simulink model "MPC_Demo_wuguzhang"  (R2024a)
settings: Solver=ode1  StartTime=0.001  StopTime=16  FixedStep=0.001  RelTol=1e-3  EnableMultiTasking=on
model workspace (MAT data in the model file):
  cc = 10
libraries: simulink x3, SignalEditorBlockLib x3, Solver_SF x1, slpidlib x1
(part 2 of 5)

== matlab function MPC_Demo_wuguzhang/区域判断1 ==
  data: sw_angle input; p output; Vx input; beta input; gamma input; miu input
function p = fcn(sw_angle,Vx,beta,gamma,miu)

% C_f=40000;
% C_r=20000;
lr=1.77;
lf=1.18;
Vx_kmh=Vx*3.6;

% Fzf=[0;0;9189.11975037333;9172.89257753388;9169.68008357533;9165.55231050759;9162.51747484095;9160.32031595229;9158.75222397292;9157.63263879663;9156.84242792417;9156.29644556306;9155.92973689187;9155.69322948405;9155.55028107646;9155.47384213415;9155.44421866605;9155.44718649260;9155.47376083021;9155.51788673978;9155.57328214499;9155.63578699923;9155.70821860851;9155.79301339052;9155.88381033351;9155.98423671869;9156.10165075385;9156.23162481467;9156.37616900971;9156.53995716690;9156.71946775849;9156.91602789466;9157.12977373991;9157.35900177799;9157.60378219249;9157.86346416105;9158.13839882949;9158.42758221491;9158.73205404812;9159.05085089054;9159.38485484332;9159.73388891475;9160.09791812571;9160.47713321269;9160.87091175547;9161.27924352332;9161.70131428228;9162.13670893715;9162.25119465208;9162.13371328829;9161.89662615060;9161.62072375802;9161.33377453683;9161.04645701186;9160.75923094872;9160.46913747053;9160.17329178094;9159.86952112061;9159.55619409438;9159.23208125106;9158.89597349374;9158.54671051215;9158.18317131761;9157.80365969706;9157.40862740084;9156.99490198417;9156.56327403121;9156.11090145246;9155.63836107854;9155.14304181031;9154.62545480688;9154.08309726592;9153.51655030897;9152.92339701533;9152.30445793787;9151.65734267787;9150.98324954037;9150.27978025100;9149.54849401502;9148.78705724291;9147.99749395029;9147.17811861429;9146.32961364023;9145.45222801732;9144.54635863102;9143.61254361701;9142.65145880786;9141.66391856333;9140.65087156101;9139.61340091796;9138.55272737068;9137.47019719979;9136.36728195278;9135.24557639213;9134.10679464885;9132.95276535214;9131.78542545848;9130.60681291198;9129.41905838467;9128.22437631368;9127.02505541532;9125.82344880873;9124.62196384518;9123.42305173582;9122.22919703789;9121.04290705517;9119.86670121392;9118.70310047333;9117.55461682614;9116.42374294949;9115.31294206332;9114.22463805584;9113.16120593367;9112.12496265589;9111.11815828058;9110.14296797516;9109.20148309344;9108.29570325586;9107.42753496328;9106.59878144358;9105.81113825995;9105.06619296821;9104.36542108858;9103.71017329634;9103.10168068776;9102.54106265282;9102.02931649768;9101.56731008034;9101.15578484112;9100.79535664774;9100.48651655602;9100.22963286796;9100.02495349837;9099.87260912941;9099.77261648909;9099.72488180259;9099.72920483449;9099.78528310230;9099.89271638063;9100.05100973315;9100.25957652591;9100.51775136266;9100.82479407640;9101.17988031029;9101.58212250571;9102.03058084126;9102.52426045332;9103.06075471025;9103.64370422649;9104.26457543072;9104.93002708322;9105.63124691432;9106.37437100819;9107.15094651253;9107.96665440744;9108.81336807313;9109.69633445555;9110.60777947923;9111.55254145516;9112.52320089777;9113.52418176325;9114.54846792220;9115.60006418080;9116.67234390949;9117.76897492153;9118.88365981330;9120.01975610293;9121.17132428400;9122.33998674980;9123.52500108388;9124.72237568611;9125.93215381899;9127.15390332978;9128.38461103408;9129.62389099137;9130.87122370054;9132.12396531067;9133.38165009435;9134.64240765836;9135.90823350735;9137.17381262979;9138.43979174581;9139.70426262269;9140.96929870188;9142.23006494317;9143.48702667105;9144.73848574261;9145.98490768102;9147.22620961346;9148.45832757067;9149.68193891794;9150.89540854279;9152.09946692694;9153.29250599965;9154.47524214457;9155.64392027933;9156.79931743560;9157.94003328539;9159.06683475530;9160.17836662401;9161.27400846420;9162.35316405762;9163.41667369569;9164.46114963219;9165.48683718486;9166.49460406433;9167.48332197006;9168.45255147890;9169.40187995365;9170.33091814691;9171.23929918847;9172.12667931283;9172.99353321036;9173.83795252978;9174.66047227625;9175.46084439008;9176.23884184991;9176.99425947219;9177.72691520493;9178.43595483914;9179.12262947800;9179.78775597519;9180.42796178708;9181.04481343585;9181.63824556895;9182.20755918311;9182.75411826632;9183.27726127969;9183.77854173865;9184.25494709212;9184.70807679673;9185.13727621803;9185.54416187298;9185.92808386959;9186.29065183294;9186.62907454713;9186.94433319175;9187.23796977694;9187.50952263651;9187.75920730937;9187.98901688782;9188.19487111912;9188.38038274938;9188.54501377853;9188.68905445379;9188.81384810983;9188.91755169024;9189.00155950188;9189.06618384626;9189.11259937906;9189.13946073346;9189.14794628887;9189.13777628342;9189.11241925098;9189.06795546235;9189.00591324040;9188.92803550922;9188.83593797253;9188.72549058666;9188.60040007013;9188.46041109369;9188.30721576260;9188.13868024649;9187.95652438225;9187.76200554478;9187.55387371407;9187.33339566974;9187.10187600015;9186.85798595093;9186.60301610154;9186.33827662843;9186.06246166969;9185.77687505833;9185.48285111761;9185.17902474031;9184.86671645031;9184.54728243101;9184.21926626098;9183.88400875977;9183.54288558470;9183.19434768002;9182.83975307511;9182.48047516083;9182.11489803783;9181.74437300424;9181.37027212888;9180.99094051592;9180.60771723464;9180.22197383280;9179.83198942762;9179.43909316975;9179.04464519644;9178.64685368611;9178.24704018468;9177.84652586583;9177.44353101682;9177.03934194044;9176.63526006740;9176.22946421814;9175.82321710509;9175.41779274990;9175.01133490472;9174.60507199669;9174.20025561793;9173.79497783479;9173.39043897471;9172.98781436236;9172.58523160036;9172.18385145352;9171.78483222679;9171.38629055754;9170.98934733794;9170.59512425417;9170.20173019505;9169.81024293323;9169.42175227098;9169.03433822826;9168.64903632711;9168.26688964956;9167.88600168867;9167.50737979472;9167.13201721731;9166.75801042809;9166.38634069489;9166.01795707694;9165.65098831136;9165.28636482660;9164.92498950869;9164.56500257735;9164.20729114031;9163.85117555379;9163.49995856455;9163.14888329486;9162.79931465538;9162.45246841663;9162.10961063919;9161.76615961809;9161.42524065759;9161.08616205752;9160.75011593112;9160.41447232285;9160.08043677145;9159.74791445801;9159.41784315397;9159.08807917760;9158.75952929936;9158.43209805246;9158.10662407759;9157.78114574669;9157.45647746913;9157.13252640769;9156.80853871300;9156.48758760731;9156.16513450298;9155.84296308772;9155.52033600389;9155.19837927131;9154.87810953021;9154.55589284817;9154.23337689272;9153.90973645886;9153.58628582371;9153.26377321609;9152.93891419752;9152.61317219732;9152.28578068594;9151.95795132814;9151.62889927955;9151.30022042890;9150.96837311411;9150.63438938231;9150.29932776197;9149.96251182374;9149.62384014353;9149.28321573536;9148.94220552383;9148.59676407268;9148.24970801778;9147.90031079378;9147.54849820835;9147.19418663520;9146.83729479511;9146.47774426855;9146.11483883250;9145.75147593996;9145.38349127999;9145.01255952511;9144.63860308171;9144.26156093720;9143.88137876192;9143.49799157288;9143.11077307682;9142.72085029774;9142.32759202698;9141.93096241681;9141.53092481218;9141.12743926432;9140.72211385775;9140.31162106930;9139.89759825382;9139.48002519135;9139.05888807827;9138.63359574431;9138.20530623938;9137.77342355425;9137.33794227599;9136.89885924561;9136.45617769900;9136.00990311330;9135.56004461712;9135.10661820550;9134.64964122897;9134.18913342764;9133.72511700914;9133.25760820384;9132.78663477521;9132.31222436749;9131.83441454675;9131.35324551806;9130.86876037535;9130.38100782374;9129.88949750568;9129.39532089785;9128.89767239263;9128.39670570991;9127.89251075950;9127.38515867153;9126.87471470855;9126.36124182622;9125.84537302540;9125.32417674066;9124.80204764373;9124.27717816046;9123.74965497105;9123.21956094014;9122.68698172171;9122.15058096026;9121.61331428066;9121.07383337722;9120.53223878927;9119.98862662081;9119.44131266172;9118.89448204180;9118.34540452371;9117.79470405791;9117.24248651038;9116.68696570384;9116.13204961098;9115.57650717806;9115.01929674752;9114.46110878973;9113.90003681558;9113.34024166399;9112.78030216564;9112.21931817364;9111.65617063807;9111.09438680595;9110.53288701850;9109.96907858246;9109.40713037513;9108.84544224835;9108.28296668101;9107.72215338406;9107.16196700390;9106.60068042785;9106.04271273031;9105.48506973811;9104.92661874766;9104.37123056312;9103.81779654349;9103.26315877928;9102.71196194787;9102.16289102456;9101.61305434381;9101.06702030360;9100.52343786971;9099.97935565814;9099.43942643879;9098.90226289252;9098.36486096320;9097.83196152604;9097.30211824824;9096.77228000188;9096.24727659962;9095.72561917264;9095.20420159652;9094.68793366034;9094.17529015220;9093.66310946008;9093.15638101205;9092.65354286529;9092.15137876786;9091.65495604354;9091.16267581500;9090.67126815681;9090.18587652965;9089.70486518508;9089.22491013787;9088.75123153871;9088.28215652445;9087.81430271343;9087.35297322559;9086.89645093644;9086.44128776102;9085.99289157789;9085.54949706705;9085.10758108635;9084.67265447228;9084.24290947923;9083.81477096228;9083.39381937667;9082.97821026826;9082.56432062449;9082.15779895098;9081.75676432518;9081.35754565497;9080.96585927416;9080.57978771574;9080.19561128358;9079.81911567907;9079.44834603789;9079.07953403780;9078.71853499425;9078.36335653528;9078.01018133438;9077.66493539057;9077.32381156977;9076.98917087538;9076.65808555041;9076.33475846475;9076.01438207727;9075.70120182675;9075.39221944393;9075.08984879800;9074.79106329829;9074.50016648975;9074.21221493326;9073.93156371471;9073.65510415465;9073.38533279459;9073.11911588335;9072.86086168176;9072.60551250247;9072.35750232993;9072.11362885112;9071.87645854419;9071.64276066227;9071.41703338043;9071.19409503255;9070.97891328353;9070.76668725115;9070.56220363977;9070.36062213141;9070.16676623038;9069.97575309295;9069.79244326532;9069.61191177581;9069.43905674777;9069.26891513290;9069.10642290637;9068.94657150124;9068.79433214199;9068.64465406892;9068.50254538053;9068.36291401772;9068.23080534635;9068.10108627381;9067.97888942288;9067.85902254783;9067.74658937943;9067.63636291736;9067.53349800935;9067.43273609398;9067.33927328873;9067.24781282018;9067.16358810446;9067.08126261596;9067.00610631782;9066.93274315734;9066.86647970992;9066.80190037374;9066.74434910862;9066.68837143878;9066.63934766640;9066.59178496736;9066.55109985993;9066.51176173381;9066.47922312323;9066.44791627699;9066.42332928407;9066.39985700145;9066.38302343676;9066.36718610350;9066.35790536529;9066.34949898786;9066.34756509533;9066.34637995183;9066.35158630174;9066.35742264984;9066.36956516410;9066.38221819143;9066.40109131636;9066.42035472158;9066.44575137466;9066.47141788195;9066.50313069284;9066.53499326668;9066.57281462646;9066.61066580000;9066.65438814625;9066.69802067264;9066.74743681868;9066.79664895074;9066.85157073368;9066.90614847950;9066.96635613957;9067.02610272506;9067.09139120889;9067.15610052285;9067.22626524970;9067.29573416449;9067.37057298801;9067.44460075050;9067.52391389544;9067.60230183596;9067.68589151065;9067.76844305329;9067.85611423211;9067.94263625370;9068.03419653442;9068.12449811267;9068.21975775248;9068.31365072647;9068.41242282498;9068.50972190681;9068.61182246135;9068.71234485189;9068.81759280996;9068.92115997967;9069.02937802419;9069.13581462855;9069.24682393678;9069.35594170585;9069.46956122092;9069.58118996668;9069.69725354845;9069.81123490420;9069.92958647542;9070.04576663818;9070.16625351992;9070.28448141173;9070.40695390077;9070.52708159548;9070.65139339837;9070.77327656374;9070.89928507917;9071.02278247981;9071.15034838708;9071.27532323693;9071.40431155569;9071.53063096107;9071.66091048074;9071.78844521701;9071.91988854349;9072.04851324764;9072.18099685385;9072.31058948489;9072.44399338367;9072.57443651075;9072.70864513503;9072.83982528940;9072.97472688172;9073.10653427471;9073.24202088877;9073.37434956707;9073.51031708560;9073.64306427034;9073.77941195981;9073.91247963514;9074.04911122048;9074.18240497941;9074.31922778111;9074.45265682371;9074.58958182582;9074.72305896922;9074.86000070964;9074.99344173365;9075.13031811045;9075.26364356886;9075.40037659979;9075.53351018252;9075.67002526166;9075.80289412797;9075.93912007685;9076.07165457506;9076.20762618958;9076.33994012781;9076.47560522790;9076.60750110780;9076.74269177696;9076.87405940493;9077.00869981931;9077.13947884137;9077.27351545784;9077.40365414580;9077.53703613674;9077.66648498117;9077.79916388242;9077.92787572113;9078.05980564928;9078.18773600171;9078.31887390679;9078.44598098113;9078.57628584215;9078.70253608326;9078.83198787754;9078.95735993264;9079.08592452977;9079.21037669982;9079.33800991224;9079.46149782897;9079.58815614573;9079.71063706644;9079.83627936397;9079.95771447561;9080.08230305370;9080.20265591840;9080.32615539886;9080.44539183517;9080.56776914034;9080.68585697589;9080.80708096845;9080.92399036489;9081.04403263091;9081.15973660608;9081.27857087922;9081.39304428237;9081.51064642570;9081.62386109856;9081.74019977021;9081.85211637016;9081.96716927885;9082.07778298625;9082.19153551012;9082.30083079064;9082.41326723261;9082.52122888913;9082.63233484261;9082.73894957698;9082.84871271454;9082.95396916875;9083.06237901625;9083.16626764384;9083.27331545418;9083.37582836775;9083.48150700280;9083.58263788106;9083.68694172124;9083.78668576590;9083.88961072053;9083.98796456124;9084.08950789954;9084.18646951440;9084.28662984099;9084.38219852528;9084.48097572667;9084.57515202541;9084.67254720946;9084.76533286020;9084.86134832245;9084.95274627654;9085.04738543560;9085.13739964485;9085.23066696680;9085.31930244827;9085.41120340674;9085.49846616097;9085.58900718734;9085.67490414514;9085.76409258794;9085.84863184481;9085.93646886810;9086.01964538010;9086.10613686697;9086.18797089807;9086.27314322536;9086.35366422064;9086.43754838884;9086.51678787281;9086.59941572272;9086.67740577499;9086.75880971112;9086.83558287214;9086.91579577764;9086.99138515247;9087.07044043382;9087.14500187794;9087.22323484432;9087.29693513225;9087.37417232406;9087.44680699600;9087.52298219243;9087.59455176603;9087.66968800239;9087.74022856174;9087.81436459954;9087.88391378967;9087.95708605231;9088.02567941450;9088.09792271657;9088.16559735393;9088.23694947224;9088.30374016880;9088.37423617995;9088.44017874072;9088.50985445681;9088.57498463890;9088.64387583344;9088.70822931438;9088.77637162225;9088.83998393678;9088.90741285284;9088.97031940026;9089.03707028063;9089.09930631883;9089.16541436883;9089.22701499811;9089.29251525340;9089.35351539604;9089.41844270236;9089.47887708251;9089.54326607469;9089.60316919797;9089.66705428081;9089.72646041517;9089.78987574472;9089.84881890290;9089.91179836935;9089.97031229242;9090.03288950432;9090.09100750218;9090.15321434384;9090.21097115970;9090.27284644192;9090.33026914247;9090.39182317885;9090.44891415001;9090.51014531504;9090.56690107222;9090.62780504086;9090.68422110941;9090.74479309351;9090.80086462530;9090.86109944684;9090.91682119582;9090.97671329867;9091.03207967777;9091.09162320377;9091.14662836125;9091.20581721828;9091.26045509588;9091.31928300664;9091.37354738122;9091.43200792080;9091.48589243780;9091.54397906436;9091.59747726662;9091.65518334896;9091.70828852845;9091.76560556839;9091.81830591656;9091.87521882074;9091.92749726091;9091.98398726991;9092.03582417151;9092.09187091782;9092.14324574108;9092.19882847263;9092.24972067278;9092.30481891756;9092.35520843377;9092.40980235764;9092.45966987547;9092.51374047335;9092.56306756352;9092.61659675861;9092.66536594767;9092.71833664020;9092.76694987876;9092.81989480617;9092.86808876453;9092.92050549057;9092.96810342592;9093.01989279830;9093.06684114055;9093.11798302856;9093.16427323767;9093.21475995923;9093.26038747559;9093.31020490417;9093.35514452025;9093.40429134211;9093.44857733735;9093.49710665222;9093.54080156992;9093.58878030276;9093.63195246381;9093.67944948780;9093.72216778626;9093.76925233330;9093.81158607260;9093.85832780560;9093.90034668310;9093.94681556859;9093.98858948693;9094.03485559718;9094.07645448033;9094.12258783019;9094.16408147988;9094.21015189685;9094.25160987319;9094.29768688632;9094.33917840403;9094.38533114412;9094.42692497715;9094.47322208532;9094.51498647982;9094.56149602333;9094.60349861659;9094.65028801027;9094.69259575552;9094.73973168868;9094.78241078507;9094.82995915415;9094.87307498192;9094.92110082739;9094.96471788756;9095.01328533645;9095.05746719566;9095.10663934031;9095.15144003416;9095.20126893841;9095.24674737198;9095.29729535224;9095.34351519106;9095.39484330569;9095.44186483479;9095.49403270614;9095.54191474796;9095.59498057768;9095.64378135122;9095.69780310035;9095.74757321444;9095.80262426398;9095.85346960418;9095.90961633900;9095.96153288463;9096.01873234039;9096.07165850125;9096.12984089964;9096.18370484932;9096.24279784089;9096.29752785857;9096.35745944501;9096.41298386023;9096.47368188364;9096.52992880802;9096.58880713305;9096.65073967242;9096.70769439850;9096.76772095231;9096.82773074806;9096.88825284891;9096.94905505763;9097.01073497949;9097.07251929632;9097.13478843100;9097.19693679578;9097.25948367104;9097.32184484524;9097.38457525148;9097.44708384530;9097.50993841479;9097.57253255286;9097.63544655280;9097.69805993309;9097.76096667378;9097.82353290400;9097.88636657838;9097.94882050614;9098.01151660772;9098.07379435580;9098.13628961984;9098.19832854112;9098.26056093330;9098.32229962355;9098.38420836398;9098.44558668810;9098.50711227660;9098.56807139169;9098.62915562766;9098.68963800023;9098.75022406668;9098.81018158530;9098.87017361564;9098.92942839833;9098.98869396987;9099.04723669124;9099.10584197675;9099.16377331364;9099.22183299192;9099.27927129301;9099.33690302033;9099.39396438344;9099.45128308826;9099.50808158991;9099.56520077116;9099.62184930654;9099.67888128045;9099.73549144172;9099.79254707600;9099.84922886866;9099.90641732850;9099.96327895499;9100.02070751691;9100.07785521032;9100.13562911006;9100.19316699408;9100.25138929539;9100.30941926024;9100.36818890428;9100.42680316664;9100.48620976831;9100.54550306141;9100.60564528441;9100.66571497179;9100.72668779054;9100.78762729948;9100.84952265743;9100.91142230118;9100.97432906924;9101.03727621998;9101.10128037666;9101.16535951998;9101.23054415542;9101.29583688059;9101.36228218336;9101.42886717296;9101.49665042266;9101.56460344714;9101.63379901040;9101.70319290551;9101.77386569885;9101.84479342531;9101.91709425770;9101.99008630599;9102.06505288356;9102.14052236799;9102.21738698952;9102.29444114421;9102.37277441748;9102.45121861840;9102.53090856501;9102.61066952746;9102.69165076241;9102.77265903962;9102.85485693570;9102.93703467206;9103.02036994155;9103.10363744838;9103.18802998038;9103.27230576112;9103.35736472043;9103.44288307748;9103.52883693248;9103.61520900346;9103.70198116388;9103.78913415925;9103.87665016692;9103.96451277306;9104.05270657283;9104.14121687553;9104.23002946061;9104.31913042516;9104.40850607472;9104.49814285144;9104.58802728667;9104.67814596862;9104.76848552049;9104.85903258592;9104.94977381980;9105.04069588332;9105.13178544139;9105.22302916288;9105.31441372175;9105.40592579971;9105.49755208934;9105.58927929796;9105.68109414329;9105.77298285200;9105.86502467816;9105.95727144182;9106.04973237141;9106.14239697193;9106.23524728144;9106.32826215611;9106.42142033773;9106.51470142641;9106.60808583706;9106.70155457438;9106.79508904889;9106.88867097361;9106.98228232267;9107.07590532060;9107.16952244378;9107.26311642400;9107.35667025140;9107.45016717604;9107.54359070953;9107.63692462611;9107.73015296389;9107.82326002584;9107.91623038111;9108.00904886616;9108.10170058562;9108.19417091310;9108.28644549212;9108.37851023637;9108.47146880858;9108.56466802631;9108.65780385781;9108.75072277300;9108.84333489244;9108.93559715681;9109.02748988741;9109.11900315649;9109.21013163942;9109.30086731147;9109.39163033542;9109.48111772913;9109.57104948012;9109.65968316338;9109.74874378270;9109.83648089723;9109.92464202773;9110.01127918637;9110.09787905307;9110.18261152622;9110.26726474740;9110.35011050194;9110.43298743615;9110.51417714731;9110.59552816735;9110.67530826991;9110.75536777396;9110.83395073786;9110.91291235638;9110.99049688588;9111.06858127637;9111.14539287131;9111.22563877390;9111.29905669339;9111.37886959546;9111.45192459170;9111.53148791288;9111.60439294497;9111.68389985308;9111.75683994196;9111.83647552279;9111.90963184981;9111.98957586428;9112.06312366376;9112.14354945137;9112.21765719014;9112.29873110822;9112.37356020120;9112.45544146430;9112.53114617726;9112.61398678338;9112.69071417765;9112.77465886385;9112.85254876679;9112.93773499093;9113.01691999048;9113.10347793543;9113.18408339511;9113.27213599184;9113.35428008229;9113.44393547413;9113.52792931658;9113.62014516006;9113.70723309837;9113.80265531428;9113.89285087622;9113.99126700142;9114.08426734551;9114.18534199452;9114.28081214436;9114.38421790520;9114.48184229974;9114.58726575906;9114.68673687684;9114.79387016483;9114.89488482556;9115.00342434748;9115.10639421280;9115.21803356981;9115.32373163035;9115.43678897280;9115.54324253492;9115.65675818817;9115.76344261149;9115.87704144072;9115.98367984075;9116.09710569349;9116.20344143075;9116.31643019831;9116.42219932338;9116.53448590031;9116.63942867321;9116.75075489222;9116.85461954785;9116.96473539559;9117.06727820176;9117.17594160895;9117.27692669389;9117.38390346947;9117.48310283418;9117.58816671721;9117.68536029751;9117.78829301737;9117.88327960229;9117.98347412535;9118.07502851036;9118.17143690609;9118.25917099087;9118.35179547629;9118.43589314209;9118.52500449886;9118.60576815830;9118.69165560934;9118.76936245151;9118.85229736205;9118.92721273233;9119.00745869867;9119.07984278309;9119.15765913235;9119.22776786027;9119.30340934826;9119.37149377519;9119.44521000035;9119.51151584834;9119.58355088318;9119.64831224611;9119.71888875423;9119.78229051408;9119.85160870726;9119.91389549335;9119.98219177510;9120.04358960801;9120.11108622362;9120.17181275648;9120.23872423264;9120.29898940402;9120.36552324501;9120.42553015671;9120.49188702999;9120.55183188481;9120.61820546563;9120.67827742679;9120.74485426263;9120.80523535575;9120.87219440930;9120.93306533647;9121.00072909876;9121.06254371323;9121.13119660006;9121.19399939212;9121.26358871951;9121.32728106362;9121.39768930015;9121.46215023415;9121.53325736777;9121.59836867986;9121.67178030971;9121.73984910651;9121.81469362973;9121.88351371954;9121.95874937738;9122.02775600253;9122.10306479959;9122.17210094333;9122.24737890456;9122.31634724850;9122.39148950185;9122.46027857939;9122.53516967457;9122.60366344609;9122.67818739912;9122.74627128960;9122.82031413911;9122.88787563093;9122.96132535402;9123.02825379265;9123.10100020894;9123.16718681728;9123.23912167433;9123.30445967306;9123.37547678109;9123.43986152745;9123.50985691118;9123.57318606083;9123.64205812697;9123.70422980378;9123.77205576467;9123.83357503584;9123.90101001834;9123.96220664999;9124.02926849033;9124.09004522663;9124.15659695408;9124.21680781094;9124.28270432164;9124.34221430027;9124.40732489533;9124.46601013781;9124.53021224465;9124.58795522831;9124.65113194922;9124.70782060935;9124.76986057280;9124.82538841670;9124.88618590817;9124.94045210389;9124.99990711147;9125.05281650636;9125.11083472382;9125.16229783854;9125.21879065283;9125.26872366139;9125.32360812590;9125.37193282203;9125.42513161584;9125.47177536483;9125.52321673922;9125.56811241775;9125.61773013030;9125.66081605520;9125.70854929406;9125.74976914095;9125.79556243961;9125.83486515374;9125.87866829781;9125.91600957773;9125.95724044050;9125.99121170212;9126.02863406286;9126.05880952445;9126.09248847543;9126.11915976076;9126.14947154751;9126.17303182736;9126.20225198389;9126.22570572409;9126.25328347015;9126.27467170389;9126.29996561425;9126.31912378599;9126.34226058284;9126.35947903220;9126.38081487214;9126.39646462860;9126.41635068636;9126.43076450956;9126.44952486201;9126.46301767558;9126.48096294433;9126.49383856383;9126.51126878215;9126.52382043261;9126.54102472172;9126.55353459729;9126.57079085190;9126.58352993698;9126.60110473528;9126.61433276200;9126.63248134612;9126.64644678611;9126.66541306394;9126.68035178511;9126.70036437828;9126.71649071401;9126.73774179251;9126.75574048307;9126.77987819052;9126.80136052105;9126.82900924986;9126.85387895669;9126.88465355073;9126.91240776485;9126.94576558247;9126.97587238470;9127.01129366991;9127.04324860163;9127.08023361112;9127.11354567678;9127.15160508012;9127.18579263687;9127.22444687146;9127.25903858875;9127.29781912561;9127.33235511139;9127.37080533606;9127.40483782437;9127.44251359894;9127.47560743645;9127.51207753775;9127.54676594504;9127.57718616582;9127.61008008743;9127.64290480880;9127.66923857515;9127.69967676543;9127.72773677794;9127.75114364276;9127.77724978939;9127.80023723094;9127.81889873591;9127.83988425756;9127.85752304349;9127.87069694655;9127.88553472756;9127.89582456812;9127.90039207691;9127.90554695929;9127.90618503260;9127.90158294790;9127.89793107813;9127.89037313121;9127.87824970114;9127.86745126833;9127.85337373552;9127.83536292616;9127.81905521835;9127.80002817102;9127.77768057028;9127.75741363961;9127.73496560112;9127.70978324736;9127.68703483868;9127.66262367966;9127.63604318570;9127.61224518740;9127.58881353361;9127.56772391919;9127.54356463785;9127.52263970230;9127.50331849746;9127.48456391293;9127.46178080594;9127.44463156975;9127.42845299543];
% Fzr=[0;0;6232.32629550717;6232.54307244978;6232.91477815521;6233.38563710747;6233.94240655566;6234.56612275444;6235.24014158343;6235.94975524797;6236.68217071639;6237.42636579874;6238.17293314253;6238.91390615096;6239.64258162136;6240.35335056316;6241.04153634985;6241.70324950225;6242.33525801826;6242.93488221073;6243.49989568850;6244.02846586667;6244.51906052474;6244.97039820592;6245.38136911708;6245.75100642514;6246.07846322588;6246.36297904621;6246.60383072906;6246.80036960347;6246.95199291188;6247.05809998131;6247.11813893918;6247.13156377948;6247.09785388636;6247.01652293840;6246.88710479195;6246.70917748785;6246.48234777519;6246.20626625045;6245.88062684790;6245.50516874294;6245.07968149210;6244.60399953319;6244.07800389371;6243.50162311781;6242.87482889067;6242.19763616486;6241.47010421653;6240.69325749782;6239.86887047308;6238.99853701667;6238.08364264689;6237.12533656300;6236.12455959022;6235.08210871880;6233.99868966421;6232.87495516622;6231.71153506660;6230.50905763089;6229.26816569714;6227.98952991147;6226.67385848920;6225.32190441570;6223.93447020719;6222.51241822826;6221.05667963157;6219.56826230537;6218.04825802087;6216.49784870904;6214.91831146876;6213.31102320262;6211.67746371988;6210.01921840042;6208.33797977737;6206.63554855827;6204.91383349772;6203.17485035373;6201.42072042279;6199.65366783259;6197.87601594993;6196.09018298240;6194.29867649363;6192.50408715584;6190.70908153284;6188.91639406113;6187.12881866016;6185.34920076739;6183.58043063022;6181.82543772309;6180.08718398131;6178.36865294418;6176.67283452149;6175.00270757929;6173.36122316766;6171.75129009974;6170.17576309679;6168.63743273341;6167.13901626998;6165.68314878347;6164.27237436612;6162.90913737779;6161.59577384296;6160.33450311111;6159.12741990012;6157.97648683183;6156.88352755229;6155.85022051378;6154.87809348015;6153.96851880348;6153.12270950579;6152.34171619001;6151.62642479179;6150.97755598273;6150.39566203877;6149.88112879779;6149.43417657454;6149.05486469573;6148.74309027663;6148.49862455822;6148.32109516155;6148.20994913313;6148.16450785900;6148.18398907915;6148.26733216398;6148.41341271497;6148.62099076394;6148.88871686543;6149.21513895527;6149.59870939931;6150.03779222830;6150.53067144950;6151.07555547907;6151.67058539835;6152.31384611903;6153.00337003910;6153.73714659725;6154.51312451647;6155.32922586525;6156.18334687456;6157.07336607688;6157.99715026078;6158.95256019230;6159.93759583914;6160.95016315556;6161.98819906054;6163.04965966232;6164.13250628364;6165.23479089180;6166.35433364972;6167.48900944461;6168.63677935195;6169.79565436234;6170.96368243236;6172.13896926358;6173.31967359229;6174.50400719840;6175.69023494123;6176.87667516223;6178.06170505400;6179.24374582456;6180.42127639731;6181.59284071226;6182.75703800449;6183.91252366763;6185.05801005314;6186.19232015262;6187.31449596826;6188.42344096218;6189.51819705809;6190.59783935364;6191.66147534015;6192.70824818866;6193.73746774156;6194.74808164146;6195.73917056629;6196.70993629329;6197.65964820737;6198.58764042383;6199.49330867453;6200.37610767006;6201.23554866657;6202.07119730098;6202.88267141960;6203.66963908356;6204.43181665521;6205.16896713034;6205.88089828291;6206.56746105420;6207.22854790898;6207.86409122286;6208.47406187048;6209.05852403975;6209.61775614362;6210.15184926026;6210.66102424303;6211.14551327852;6211.60555333665;6212.04139013678;6212.45328440392;6212.84155312069;6213.20654460609;6213.54818451946;6213.86668640068;6214.16229575237;6214.43529544672;6214.68600186793;6214.91476162182;6215.12194859209;6215.30796126885;6215.47322036576;6215.61816664606;6215.74325886941;6215.84897195107;6215.93579520111;6216.00423089911;6216.05479273188;6216.08800523180;6216.10439905011;6216.10451413064;6216.08889765087;6216.05810244017;6216.01275759639;6215.95361368156;6215.88121559152;6215.79621429256;6215.69924316657;6215.59091770681;6215.47183771977;6215.34258908201;6215.20374627649;6215.05586918862;6214.89965852940;6214.73545381670;6214.56360571013;6214.38456114853;6214.19877595683;6214.00671218816;6213.80883540318;6213.60561253909;6213.39751008011;6213.18499242210;6212.96852054834;6212.74855080405;6212.52553404491;6212.29991470726;6212.07213000898;6211.84260932788;6211.61177358329;6211.38003468928;6211.14779503167;6210.91544696403;6210.68337256638;6210.45194316022;6210.22151902998;6209.99246020095;6209.76532049044;6209.54036367215;6209.31796855286;6209.09849329397;6208.88227042621;6208.66960906184;6208.46079678628;6208.25610126088;6208.05577161734;6207.86003958897;6207.66912039667;6207.48334009407;6207.30278886318;6207.12744366031;6206.95740495393;6206.79277311370;6206.63364715094;6206.48012346085;6206.33229481613;6206.19024963394;6206.05407159773;6205.92383925885;6205.79962581958;6205.68149914694;6205.56952166886;6205.46375038059;6205.36423695986;6205.27102775488;6205.18416394500;6205.10368174323;6205.02961240169;6204.96198242721;6204.90081388743;6204.84612444751;6204.79792752491;6204.75640587035;6204.72153470589;6204.69334033636;6204.67186727776;6204.65714568721;6204.64919341197;6204.64801780378;6204.65361693010;6204.66598083127;6204.68509275114;6204.71092991295;6204.74346222326;6204.78265904750;6204.82853175901;6204.88115179724;6204.94020928045;6205.00561803686;6205.07729616520;6205.15516841437;6205.23916465508;6205.32921878341;6205.42526809591;6205.52725250011;6205.63511397390;6205.74879629675;6205.86824459694;6205.99340496484;6206.12422447159;6206.26065087089;6206.40263250683;6206.55011830475;6206.70305765397;6206.86139991053;6207.02509507597;6207.19409348994;6207.36834579852;6207.54780278749;6207.73253047355;6207.92249492935;6208.11763883793;6208.31795073179;6208.52341070259;6208.73399190606;6208.94966184019;6209.17038339978;6209.39611572623;6209.62681502371;6209.86243513669;6210.10292801924;6210.34824426433;6210.59833324054;6210.85314375951;6211.11262415044;6211.37680024137;6211.64563275382;6211.91889712103;6212.19651273494;6212.47840530174;6212.76450670357;6213.05475415533;6213.34908918386;6213.64745348996;6213.94980192073;6214.25608177929;6214.56624613090;6214.88024984879;6215.19804927543;6215.51960207411;6215.84486702092;6216.17380395790;6216.50637360705;6216.84253743073;6217.18225755812;6217.52549661361;6217.87221777134;6218.22238457463;6218.57596079207;6218.93291029659;6219.29333120175;6219.65712566143;6220.02428343472;6220.39479307441;6220.76863697282;6221.14579243785;6221.52623254301;6221.90992684291;6222.29684187085;6222.68694153615;6223.08018756314;6223.47653983935;6223.87595670669;6224.27839346810;6224.68380823475;6225.09215639671;6225.50339129141;6225.91746635481;6226.33433376693;6226.75394475990;6227.17639939794;6227.60145517817;6228.02903561687;6228.45907232249;6228.89150075567;6229.32625944927;6229.76328931003;6230.20253303801;6230.64393463598;6231.08743904390;6231.53299179711;6231.98053890938;6232.43002665144;6232.88140140623;6233.33460955766;6233.78959736315;6234.24631086481;6234.70469575265;6235.16469738838;6235.62626071425;6236.08933015638;6236.55384966182;6237.01976267974;6237.48701215796;6237.95554053729;6238.42528970225;6238.89628911481;6239.36844916086;6239.84171937130;6240.31605699245;6240.79141452918;6241.26774000497;6241.74497774611;6242.22306900801;6242.70195006769;6243.18155353923;6243.66180950138;6244.14264587439;6244.62398889832;6245.10576349998;6245.58789362644;6246.07030256871;6246.55291324194;6247.03564826367;6247.51843002977;6248.00118084498;6248.48382300004;6248.96627882496;6249.44847078858;6249.93032142681;6250.41175333223;6250.89272200385;6251.37318787692;6251.85296928028;6252.33197760981;6252.81012691231;6253.28733434283;6253.76351960102;6254.23860456611;6254.71251292996;6255.18516994540;6255.65650230787;6256.12643798495;6256.59490618762;6257.06183723674;6257.52716244149;6257.99081412096;6258.45272452139;6258.91282390173;6259.37104244001;6259.82731019489;6260.28155752044;6260.73371515528;6261.18371458789;6261.63148827798;6262.07696955473;6262.52009287576;6262.96079393272;6263.39900953590;6263.83471509219;6264.26786614187;6264.69838981181;6265.12624084926;6265.55137213252;6265.97373512237;6266.39328053268;6266.80995873773;6267.22371991912;6267.63451452720;6268.04229350587;6268.44700828650;6268.84861118627;6269.24705538980;6269.64229499736;6270.03428526246;6270.42298257896;6270.80834446780;6271.19032977736;6271.56889863779;6271.94401241881;6272.31563391109;6272.68372725921;6273.04825790343;6273.40919274914;6273.76650008666;6274.12014952336;6274.47011214560;6274.81636043000;6275.15886816665;6275.49761061829;6275.83256442392;6276.16370752940;6276.49101932996;6276.81448060413;6277.13407345579;6277.44984826445;6277.76171274427;6278.06963857261;6278.37360695119;6278.67360203923;6278.96961111902;6279.26162348542;6279.54963035640;6279.83362470823;6280.11360125645;6280.38955625502;6280.66148735875;6280.92939369905;6281.19327571323;6281.45313503489;6281.70897459717;6281.96079847795;6282.20861180562;6282.45242087643;6282.69223300835;6282.92805645465;6283.15990052961;6283.38777546617;6283.61169233613;6283.83166319343;6284.04770080793;6284.25981889731;6284.46803187985;6284.67235502283;6284.87280422751;6285.06941331865;6285.26221716409;6285.45122125625;6285.63645173386;6285.81793359921;6285.99569077622;6286.16974663266;6286.34012390789;6286.50684520593;6286.66993287453;6286.82940930867;6286.98529683282;6287.13761802172;6287.28639544274;6287.43165198542;6287.57341065358;6287.71169477161;6287.84652780797;6287.97793358862;6288.10593608951;6288.23055965142;6288.35182876148;6288.46976826484;6288.58440314260;6288.69575871935;6288.80386042444;6288.90873400216;6289.01040528240;6289.10890039295;6289.20424553008;6289.29646717135;6289.38559184397;6289.47164633870;6289.55465747187;6289.63465220569;6289.71165746974;6289.78570043891;6289.85680830099;6289.92500847689;6289.99032838028;6290.05279563342;6290.11243782368;6290.16928272419;6290.22335805077;6290.27469168612;6290.32331143623;6290.36924525640;6290.41252100906;6290.45316669306;6290.49121019948;6290.52667954363;6290.55960261971;6290.59000758036;6290.61792222515;6290.64337423408;6290.66639118118;6290.68700070156;6290.70523027147;6290.72110746011;6290.73466290452;6290.74595376259;6290.75496624998;6290.76172479797;6290.76625415103;6290.76857984531;6290.76872782054;6290.76672455514;6290.76259671958;6290.75637135298;6290.74807554510;6290.73773664073;6290.72538194170;6290.71103892849;6290.69473497384;6290.67649757655;6290.65635408265;6290.63433192725;6290.61045836024;6290.58476069396;6290.55726608694;6290.52800164533;6290.49699435946;6290.46427110637;6290.42985865268;6290.39378364350;6290.35607260431;6290.31675193173;6290.27584789545;6290.23338662897;6290.18939413225;6290.14389626197;6290.09691873331;6290.04848711201;6289.99862681723;6289.94736311254;6289.89472111094;6289.84072576600;6289.78540187655;6289.72877407842;6289.67086684948;6289.61170450082;6289.55131118206;6289.48971087131;6289.42692738282;6289.36298435750;6289.29790526964;6289.23171341796;6289.16443193315;6289.09608946626;6289.02671521977;6288.95632698547;6288.88494971010;6288.81260756095;6288.73932400563;6288.66512190818;6288.59002361436;6288.51405101500;6288.43722560424;6288.35956852014;6288.28110058455;6288.20184232814;6288.12181401907;6288.04103567767;6287.95952709623;6287.87730784891;6287.79439730641;6287.71081464059;6287.62657883582;6287.54170869023;6287.45622282519;6287.37013968454;6287.28347754162;6287.19625449585;6287.10848847900;6287.02019725335;6286.93139841737;6286.84210940240;6286.75234747824;6286.66212974914;6286.57147315903;6286.48039448727;6286.38891035384;6286.29703721294;6286.20479135888;6286.11218892106;6286.01924586829;6285.92597800448;6285.83240097389;6285.73853025586;6285.64438117035;6285.54996887229;6285.45530835669;6285.36041445175;6285.26530182567;6285.16998498050;6285.07447825804;6284.97879583332;6284.88295172015;6284.78695976560;6284.69083365563;6284.59458690948;6284.49823287987;6284.40178458428;6284.30525475956;6284.20865601812;6284.11200085529;6284.01530164610;6283.91857064800;6283.82181998362;6283.72506163852;6283.62830744792;6283.53156909845;6283.43485811912;6283.33818588476;6283.24156360785;6283.14500234352;6283.04851298186;6282.95210625356;6282.85579272274;6282.75958279165;6282.66348669293;6282.56751448412;6282.47167603779;6282.37598105310;6282.28043905458;6282.18505940504;6282.08985130338;6281.99482379558;6281.89998576887;6281.80534596204;6281.71091296000;6281.61669520197;6281.52270097453;6281.42893842088;6281.33541553385;6281.24214016406;6281.14912001262;6281.05636263775;6280.96387544931;6280.87166571557;6280.77974055655;6280.68810695194;6280.59677173309;6280.50574159073;6280.41502306644;6280.32462252283;6280.23454614690;6280.14479997278;6280.05538987084;6279.96632155992;6279.87760060292;6279.78923241860;6279.70122227596;6279.61357530482;6279.52629648856;6279.43939067409;6279.35286256555;6279.26671673308;6279.18095760586;6279.09558948113;6279.01061651689;6278.92604274095;6278.84187204314;6278.75810818491;6278.67475479055;6278.59181535654;6278.50929324396;6278.42719168821;6278.34551379083;6278.26426252938;6278.18344074960;6278.10305117463;6278.02309639763;6277.94357889133;6277.86450099967;6277.78586494736;6277.70767283147;6277.62992663216;6277.55262820455;6277.47577928850;6277.39938150098;6277.32343634598;6277.24794520649;6277.17290935492;6277.09832994447;6277.02420801956;6276.95054450656;6276.87734022285;6276.80459587694;6276.73231206936;6276.66048927789;6276.58912785949;6276.51822803484;6276.44778989298;6276.37781337833;6276.30829829829;6276.23924431109;6276.17065093583;6276.10251754240;6276.03484336233;6275.96762747938;6275.90086884084;6275.83456624897;6275.76871819920;6275.70332269923;6275.63837774298;6275.57388123595;6275.50983103520;6275.44622494243;6275.38306069719;6275.32033595544;6275.25804829134;6275.19619518114;6275.13477400952;6275.07378205688;6275.01321650643;6274.95307440552;6274.89335268587;6274.83404816198;6274.77515754311;6274.71667742726;6274.65860431509;6274.60093460263;6274.54366459507;6274.48679049893;6274.43030843573;6274.37421443391;6274.31850444249;6274.26317432256;6274.20821986106;6274.15363676203;6274.09942066030;6274.04556711275;6273.99207161192;6273.93892957688;6273.88613636724;6273.83368727372;6273.78157753202;6273.72980231344;6273.67835673868;6273.62723586854;6273.57643471739;6273.52594824390;6273.47577136461;6273.42589894426;6273.37632580988;6273.32704674028;6273.27805648116;6273.22934974096;6273.18092120742;6273.13276555093;6273.08487745157;6273.03725160201;6272.98988273380;6272.94276561580;6272.89589507562;6272.84926599378;6272.80287332236;6272.75671207613;6272.71077734880;6272.66506430281;6272.61956818385;6272.57428430938;6272.52920808268;6272.48433497985;6272.43966056376;6272.39518047041;6272.35089042227;6272.30678621437;6272.26286372733;6272.21911891313;6272.17554780820;6272.13214651861;6272.08891123305;6272.04583820836;6272.00292377693;6271.96016432695;6271.91755631405;6271.87509624666;6271.83278069923;6271.79060629860;6271.74856973777;6271.70666776237;6271.66489718446;6271.62325486870;6271.58173774555;6271.54034279711;6271.49906707032;6271.45790766225;6271.41686173290;6271.37592649028;6271.33509920335;6271.29437718666;6271.25376129659;6271.21325674296;6271.17285496884;6271.13255502899;6271.09235560243;6271.05225509759;6271.01225175727;6270.97234367883;6270.93252886056;6270.89280521203;6270.85317058796;6270.81362279045;6270.77415958630;6270.73477870423;6270.69547783496;6270.65625459909;6270.61710654071;6270.57803109363;6270.53902558097;6270.50008718961;6270.46121297648;6270.42239984851;6270.38364457410;6270.34494376645;6270.30629389807;6270.26769128659;6270.22913211127;6270.19061240011;6270.15212804831;6270.11367480581;6270.07524829671;6270.03684400788;6269.99845730846;6269.96008343935;6269.92171753269;6269.88335460157;6269.84498956030;6269.80661721370;6269.76823227761;6269.72982936841;6269.69140302334;6269.65294769033;6269.61445774811;6269.57592749597;6269.53735117401;6269.49872295257;6269.46003695284;6269.42128723557;6269.38246782215;6269.34357268304;6269.30459575839;6269.26553094686;6269.22639616321;6269.18716676098;6269.14782437929;6269.10836075743;6269.06876810558;6269.02903902178;6268.98916643421;6268.94914352666;6268.90896370843;6268.86862056025;6268.82810814584;6268.78742004619;6268.74654988618;6268.70549143248;6268.66423852249;6268.62278504707;6268.58112499840;6268.53925249409;6268.49716183830;6268.45484754418;6268.41230438232;6268.36952738691;6268.32651188998;6268.28325351548;6268.23974820507;6268.19599220470;6268.15198208483;6268.10771472277;6268.06318731914;6268.01839737926;6267.97334272089;6267.92802142481;6267.88243195987;6267.83657302047;6267.79044359248;6267.74404254163;6267.69736825140;6267.65041960255;6267.60319589310;6267.55569683391;6267.50792259171;6267.45987369186;6267.41155102878;6267.36295578563;6267.31408945722;6267.26495377970;6267.21555076160;6267.16588261908;6267.11595181103;6267.06576097763;6267.01531297771;6266.96461082963;6266.91365775063;6266.86245709870;6266.81101241325;6266.75932735831;6266.70740576405;6266.65525157035;6266.60286886927;6266.55026184942;6266.49743483852;6266.44439224844;6266.39113861798;6266.33767855883;6266.28401679810;6266.23015811482;6266.17610745062;6266.12186985349;6266.06745046485;6266.01285440660;6265.95808676506;6265.90315248829;6265.84805639209;6265.79280307937;6265.73739696317;6265.68184220050;6265.62614272608;6265.57030219549;6265.51432402612;6265.45821134590;6265.40196703873;6265.34559369759;6265.28909367301;6265.23246902838;6265.17572159093;6265.11885290852;6265.06186430194;6265.00475682277;6264.94753130700;6264.89018833293;6264.83272827562;6264.77517541802;6264.71752346223;6264.65977091773;6264.60192195165;6264.54397934321;6264.48594476488;6264.42781892011;6264.36960174224;6264.31129247283;6264.25288981136;6264.19439195338;6264.13579670755;6264.07710150720;6264.01830350624;6263.95939957309;6263.90038637201;6263.84126034594;6263.78201778792;6263.72265481620;6263.66316743977;6263.60355152764;6263.54380287035;6263.48391714580;6263.42388998595;6263.36371690219;6263.30339333629;6263.24291415181;6263.18230157418;6263.12155010616;6263.06061447383;6262.99948566888;6262.93815597893;6262.87661884862;6262.81486875200;6262.75290100432;6262.69071169388;6262.62829754305;6262.56565587848;6262.50278452259;6262.43968179594;6262.37634754298;6262.31278108416;6262.24898193827;6262.18495002186;6262.12068538995;6262.05618829470;6261.99145917929;6261.92649868517;6261.86130765314;6261.79588713032;6261.73023837047;6261.66436283090;6261.59826216851;6261.53193823391;6261.46539306524;6261.39862888154;6261.33164807564;6261.26445320717;6261.19704699564;6261.12943231355;6261.06161217944;6260.99358975144;6260.92536832053;6260.85695130410;6260.78834223979;6260.71954477934;6260.65056268231;6260.58139981049;6260.51206012192;6260.44254766556;6260.37286656640;6260.30302085490;6260.23301437752;6260.16285080973;6260.09253367361;6260.02206636792;6259.95145219567;6259.88069438498;6259.80979610436;6259.73876047454;6259.66759057694;6259.59628946008;6259.52486014451;6259.45330562613;6259.38162887912;6259.30983285746;6259.23792049664;6259.16589471422;6259.09375841049;6259.02151446863;6258.94916575504;6258.87671511918;6258.80416539325;6258.73151939255;6258.65877991475;6258.58594974021;6258.51303163151;6258.44002833355;6258.36694252093;6258.29377508372;6258.22052681016;6258.14719855508;6258.07379151729;6258.00033579600;6257.92683533752;6257.85328475756;6257.77969337212;6257.70606887251;6257.63241764065;6257.55874499085;6257.48505536380;6257.41135250652;6257.33763957118;6257.26391926075;6257.19019387382;6257.11646542047;6257.04273593874;6256.96900804130;6256.89528472683;6256.82156936869;6256.74786554081;6256.67417693346;6256.60050721413;6256.52685999703;6256.45327968724;6256.37976653188;6256.30627063168;6256.23278964525;6256.15932212628;6256.08586745744;6256.01242560079;6255.93899697208;6255.86558227439;6255.79218246333;6255.71879854776;6255.64543161505;6255.57208272250;6255.49875291733;6255.42544314964;6255.35215430944;6255.27888715228;6255.20564234633;6255.13242040684;6255.05922174997;6254.98604663282;6254.91289521194;6254.83976748696;6254.76666336148;6254.69358258941;6254.62052483730;6254.54748963205;6254.47447642415;6254.40148453631;6254.32851322686;6254.25556163896;6254.18262886428;6254.10971389175;6254.03681567136;6253.96393306347;6253.89106490278;6253.81820959224;6253.74536442604;6253.67252584675;6253.59969049341;6253.52685373359;6253.45400874680;6253.38114950577;6253.30826992533;6253.23536412252;6253.16242660245;6253.08945229295;6253.01643666231;6252.94337570550;6252.87026602530;6252.79710479200;6252.72388980375;6252.65061796532;6252.57728352499;6252.50388160929;6252.43040779806;6252.35685844727;6252.28323082791;6252.20952300147;6252.13573382559;6252.06186285553;6251.98791036248;6251.91387724685;6251.83976506696;6251.76557595879;6251.69131266717;6251.61697846823;6251.54257720246;6251.46811319894;6251.39359130913;6251.31901683308;6251.24439555394;6251.16973366545;6251.09503780731;6251.02031499340;6250.94557264812;6250.87081853522;6250.79606079464;6250.72130788476;6250.64656929842;6250.57186459856;6250.49724453050;6250.42269577640;6250.34823925527;6250.27389461505;6250.19967977830;6250.12561109225;6250.05170354864;6249.97797087554;6249.90442570806;6249.83107963803;6249.75794334902;6249.68502663851;6249.61233852926;6249.53988727288;6249.46768044597;6249.39572494172;6249.32402705536;6249.25259246823;6249.18148578411;6249.11067683111;6249.04012718220;6248.96983487982;6248.89979883299;6248.83001861353;6248.76049430138;6248.69122627961;6248.62221515488;6248.55346161217;6248.48496638189;6248.41673013279;6248.34875346980;6248.28103685211;6248.21358061114;6248.14638488445;6248.07944964701;6248.01277465638;6247.94635949156;6247.88020350545;6247.81430587031;6247.74866552833;6247.68328100491;6247.61815048528;6247.55327193381;6247.48864316703;6247.42426200793;6247.36012633006;6247.29623416966;6247.23258373471;6247.16917348780;6247.10600205896;6247.04306546816;6246.98036005101;6246.91788253400;6246.85563050429;6246.79360252262;6246.73179797108;6246.67021698829;6246.60886033268;6246.54772934508;6246.48682584302;6246.42615211103;6246.36571081532;6246.30550500861;6246.24553805539;6246.18581364525;6246.12633572526;6246.06710851825;6246.00813646063;6245.94942422434;6245.89097665797;6245.83279881145;6245.77489587953;6245.71727322815;6245.65993633712;6245.60289082666;6245.54614240136;6245.48969687611;6245.43356012172;6245.37773809208;6245.32223676423;6245.26706185460;6245.21221915753;6245.15771516265;6245.10355301750;6245.04973643576;6244.99626835034;6244.94315120492;6244.89038701381;6244.83797747982;6244.78592401749;6244.73422784170;6244.68288996896;6244.63191128799;6244.58129254682;6244.53103441172;6244.48113744517;6244.43160215684;6244.38242897545;6244.33361829459;6244.28517044092;6244.23708571609;6244.18936436242;6244.14200660305;6244.09501260557;6244.04838252071;6244.00211644547;6243.95621446033;6243.91067659209;6243.86550285051;6243.82069319094;6243.77624755042;6243.73216581058;6243.68844783304;6243.64509342286;6243.60210236378;6243.55947438133;6243.51720917850;6243.47530639916;6243.43376566306;6243.39258655858;6243.35176961919;6243.31131656345;6243.27123014270;6243.23151384722;6243.19217163671;6243.15320764119;6243.11462599106;6243.07643054709;6243.03862154957;6243.00119886826;6242.96416214070;6242.92751100077;6242.89124552098;6242.85536558838;6242.81987124963;6242.78476211298;6242.75003771520;6242.71569700706;6242.68173875165;6242.64816105061;6242.61496176395;6242.58213806047;6242.54968684810;6242.51760434061;6242.48588649298;6242.45452858104;6242.42352563752;6242.39287204137;6242.36256195332;6242.33258891219;6242.30294626811;6242.27362678487;6242.24462307024;6242.21592718251;6242.18754405276;6242.15946604679;6242.13168072572;6242.10418199784;6242.07696285127;6242.05005513092;6242.02341148260;6241.99700302656;6241.97081260203;6241.94482283814;6241.91901687717;6241.89337821371;6241.86789125383;6241.84254106062;6241.81731383184;6241.79219658705;6241.76717759462;6241.74224602500;6241.71739234393;6241.69260794518;6241.66788551944;6241.64321867566;6241.61860229232;6241.59403213254;6241.56950518274;6241.54501926564;6241.52057336867;6241.49616725816;6241.47180179942;6241.44747857267;6241.42320018361;6241.39896997049;6241.37479203109;6241.35067127434;6241.32661330584;6241.30262436348;6241.27871141725;6241.25488200706;6241.23114422485;6241.20750679467;6241.18397889029;6241.16057015758;6241.13729075553;6241.11415164200;6241.09116607899;6241.06834897359;6241.04571638914;6241.02328499495;6241.00107157523;6240.97909246018;6240.95736323232;6240.93589849854;6240.91471171325;6240.89381485797;6240.87321858606;6240.85293202066;6240.83296258522;6240.81331621681;6240.79399723080;6240.77500819053;6240.75635020160;6240.73802279270;6240.72002379126;6240.70234965851;6240.68499534902;6240.66795169927;6240.65120637074;6240.63474630328;6240.61855777230;6240.60262663825;6240.58693831134;6240.57147769154;6240.55622904970];
% 
% alpha_fy=(-0.3+0.6/1462:0.6/1462:0.3);
alpha_ry=(-0.25+0.5/1462:0.5/1462:0.25);

% %定义矩阵分配内存
% Fyfy=zeros(1,length(alpha_fy));
% Fyry=zeros(1,length(alpha_ry));
% C1=zeros(1,length(alpha_fy)-1);C3=zeros(1,length(alpha_ry)-1);
% Cfl=zeros(1,258);Crl=zeros(1,258);
% 
% 
% for iif=1:length(alpha_fy)
%     if abs(alpha_fy(iif))<atan((3*miu*Fzf(iif))/C_f)
%     Fyfy(iif)=(-C_f*alpha_fy(iif)+(C_f)^2/(3*miu*Fzf(iif))*abs(alpha_fy(iif))*alpha_fy(iif)-(C_f)^3/(27*miu^2*Fzf(iif)^2)*(alpha_fy(iif))^3);
%     else
%         Fyfy(iif)=-miu*Fzf(iif)*sign(alpha_fy(iif));
%     end
% end
% for iir=1:length(alpha_ry)
%     if abs(alpha_ry(iir))<atan((3*miu*Fzr(iir))/C_r)
%     Fyry(iir)=(-C_r*alpha_ry(iir)+(C_r)^2/(3*miu*Fzr(iir))*abs(alpha_ry(iir))*alpha_ry(iir)-(C_r)^3/(27*miu^2*Fzr(iir)^2)*(alpha_ry(iir))^3);
%     else
%          Fyry(iir)=-miu*Fzr(iir)*sign(alpha_ry(iir));
%     end
% end
% 
% for x1=1:length(alpha_fy)-1
% C1(x1)=(Fyfy(x1+1)-Fyfy(x1))/(-(alpha_fy(x1+1))-(-alpha_fy(x1)));
% Cfll=C1';
% end
% for x3=1:length(alpha_ry)-1
% C3(x3)=(Fyry(x3+1)-Fyry(x3))/(-(alpha_ry(x3+1))-(-alpha_ry(x3)));
% Crll=C3';
% end
% for aaf=1:258
%   Cfl(aaf)=Cfll(5*aaf);
% end
% for aar=1:258
%    Crl(aar)=Crll(5*aar); 
% end

alpharl=[alpha_ry];


% for i=1:a 
%         for k=1:c 
%                 if Cfl(i)>(-(lr*(Crl(k))*1430*(Vx^2)))/(2*(Crl(k))*((lf+lr)^2)-1430*(Vx^2)*lf)
%                     aa=[Cfl(i) Crl(k)];
%                     cc=[-alphafl(5*i+1) -alpharl(5*k+1)];
%                     A=[A;aa];
%                     C=[C;cc];
%                 else
%                     bb=[Cfl(i) Crl(k)];
%                     dd=[-alphafl(5*i+1) -alpharl(5*k+1)];
%                     B=[B;bb];
%                     D=[D;dd];
%                 end
%         end
% end

% Cf=B(:,1);
% Cr=B(:,2);
% osCf=[];
% osCr=[];
% oalphaf=[];
% oalphar=[];
% usCf=[];
% usCr=[];
% ualphaf=[];
% ualphar=[];
beta1_right=zeros(1,length(alpharl));
gamma1_right=zeros(1,length(alpharl));

% for p=1:length(Cf)
%     if lf*Cf(p)-lr*Cr(p)>0
%         osCf=[osCf;Cf(p)];%%婊¤冻杩囧害杞悜鏉′欢鐨凜f
%         osCr=[osCr;Cr(p)];%%婊¤冻杩囧害杞悜鏉′欢鐨凜r
%         oalphaf=[oalphaf;Alphaf(p)];%%婊¤冻杩囧害杞悜鏉′欢鐨刟lphaf
%         oalphar=[oalphar;Alphar(p)];%%婊¤冻杩囧害杞悜鏉′欢鐨刟lphar
%     else
%         usCf=[usCf;Cf(p)];%%婊¤冻涓嶈冻杞悜鏉′欢鐨凜f
%         usCr=[usCr;Cr(p)];%%婊¤冻涓嶈冻杞悜鏉′欢鐨凜r
%         ualphaf=[ualphaf;Alphaf(p)];%%婊¤冻涓嶈冻杞悜鏉′欢鐨刟lphaf
%         ualphar=[ualphar;Alphar(p)];%%婊¤冻涓嶈冻杞悜鏉′欢鐨刟lphar
%     end
% end    
kekoalphaf=-0.3;%%%%%鍜岄�鎷╃殑鍓嶈疆渚у亸瑙掔殑澶у皬鏈夊叧

%%
if Vx_kmh <= 52.5
%% 外区域
for n=1:length(alpharl)
    if abs(alpharl(n))<abs(kekoalphaf)%%鐢ㄤ笉瓒宠浆鍚戞椂鍓嶅悗杞晶鍋忚鐨勫ぇ灏忓叧绯荤瓫閫夊悎閫傜殑
    beta1_right(n)=((sw_angle-kekoalphaf)*lr-lf*alpharl(n))/(lf+lr);
    gamma1_right(n)=((sw_angle-kekoalphaf+alpharl(n))*Vx)/(lf+lr);
    end
end

   beta11_50_right_down=beta1_right(1);
   gamma11_50_right_down=gamma1_right(1);
   beta1n_50_right_up=beta1_right(length(beta1_right));
   gamma1n_50_right_up=gamma1_right(length(gamma1_right));
   
    centerx_50=beta1n_50_right_up-0.0829;
    centery_50=gamma1n_50_right_up-2.8718;
   
    beta1d1_50_left_up=2*centerx_50-beta1_right(1);
    gamma1d1_50_left_up=2*centery_50-gamma1_right(1);
    beta1dn_50_left_down=2*centerx_50-beta1_right(length(beta1_right));
    gamma1dn_50_left_down=2*centery_50-gamma1_right(length(gamma1_right));
    
g1=2.1343+gamma1dn_50_left_down;%璁＄畻ogamma2_down(1)-gamma1dn_50_left_down=锛熶綔涓哄墠闈㈢殑涓?釜鍔犳暟;
b1=0.0504+beta1dn_50_left_down;%obeta2_down(1)-beta1dn_50_left_down=锛?
g2=0.8857+g1;%ogamma2_down(length(ogamma2_down))-ogamma2_down(1)=锛?
b2=0.0993+b1;%obeta2_down(length(obeta2_down))-obeta2_down(1)=锛?
g3=2*centery_50-g1;%%-g1
b3=2*centerx_50-b1;%%-b1
g4=2*centery_50-g2;%%-g2
b4=2*centerx_50-b2;%%-b2

%x11=gamma1dn_50_left_down:0.000005:g1;
       px111_opposite =     0.02363 ;
       px112_opposite =     -0.01506;
%x12=g1:0.000005:g2;
       px121_opposite =      0.9708  ;
       px122_opposite =       1.558;
       px123_opposite =       0.811 ;
       px124_opposite =       0.2015;
       px125_opposite =       0.1418 ;
       px126_opposite =       0.03833  ;
%x13=g2:0.000005:gamma11_50_right_down;
       px131_opposite =     1.861 ;% (-5.636e+05, -2.701e+05)
       px132_opposite =     -0.2091;% (-6.956e+04, -3.484e+04)
%x21=gamma1d1_50_left_up:0.000005:g4;
       px211_opposite =         1.86 ;
       px212_opposite =       0.2089;
%x22= g4:0.000005:g3;
       px221_opposite =        0.9708 ;% (-6.388e+05, -3.304e+05)
       px222_opposite =       -1.558;% (4.151e+04, 8.218e+04)
       px223_opposite =        0.811  ;%  (-561.4, 843.6)
       px224_opposite =        -0.2015;% (-313, -264.4)
       px225_opposite =     0.1418 ;%  (18.8, 19.9)
       px226_opposite =   -0.03833  ;% (-0.3822, -0.3702)
%x23=g3:0.000005:gamma1n_50_right_up;
       px231_opposite =      0.02362 ;% (-5.636e+05, -2.701e+05)
       px232_opposite =        0.01506;% (-6.956e+04, -3.484e+04)
%x33=gamma11_50_right_down:0.000005:gamma1n_50_right_up;   
       px31_opposite =       -0.0756  ;%(-21.16, -21.16)
       px32_opposite =       0.3 ;% (2.222, 2.222)
%x44=gamma1dn_50_left_down:0.000005:gamma1d1_50_left_up; 
       px41_opposite =      -0.0756  ;%(-21.16, -21.16)
       px42_opposite =       -0.3 ;%(-2.222, -2.222)  
d3=beta11_50_right_down-px31_opposite*gamma11_50_right_down;
d4=beta1d1_50_left_up-px41_opposite*gamma1d1_50_left_up;
gamma1dn_50_0_opposite= -2.8718;
beta1dn_50_0_opposite=-0.0829;
gamma1d1_50_0_opposite=-0.2629;
beta1d1_50_0_opposite=-0.2801;       
       
oobeta1_cal_1 = px111_opposite*(gamma-(gamma1dn_50_left_down(1)-(gamma1dn_50_0_opposite))) + px112_opposite +(beta1dn_50_left_down(1)-(beta1dn_50_0_opposite));
oobeta1_cal = px121_opposite*(gamma-(gamma1dn_50_left_down(1)-(gamma1dn_50_0_opposite))).^5 + px122_opposite*(gamma-(gamma1dn_50_left_down(1)-(gamma1dn_50_0_opposite))).^4 + px123_opposite*(gamma-(gamma1dn_50_left_down(1)-(gamma1dn_50_0_opposite))).^3 + px124_opposite*(gamma-(gamma1dn_50_left_down(1)-(gamma1dn_50_0_opposite))).^2 + px125_opposite*(gamma-(gamma1dn_50_left_down(1)-(gamma1dn_50_0_opposite))) + px126_opposite+(beta1dn_50_left_down(1)-(beta1dn_50_0_opposite));
oobeta1_cal_3 = px131_opposite*(gamma-(gamma11_50_right_down(1)-(-gamma1d1_50_0_opposite))) + px132_opposite +(beta11_50_right_down(1)-(-beta1d1_50_0_opposite));
oobeta2_cal_1 = px211_opposite*(gamma-(gamma1d1_50_left_up(1)-(gamma1d1_50_0_opposite))) + px212_opposite +(beta1d1_50_left_up(1)-(beta1d1_50_0_opposite));
oobeta2_cal = px221_opposite*(gamma-(gamma1d1_50_left_up(1)-(gamma1d1_50_0_opposite))).^5 + px222_opposite*(gamma-(gamma1d1_50_left_up(1)-(gamma1d1_50_0_opposite))).^4 + px223_opposite*(gamma-(gamma1d1_50_left_up(1)-(gamma1d1_50_0_opposite))).^3 + px224_opposite*(gamma-(gamma1d1_50_left_up(1)-(gamma1d1_50_0_opposite))).^2 + px225_opposite*(gamma-(gamma1d1_50_left_up(1)-(gamma1d1_50_0_opposite))) + px226_opposite+(beta1d1_50_left_up(1)-(beta1d1_50_0_opposite));
oobeta2_cal_3 = px231_opposite*(gamma-(gamma1d1_50_left_up(1)-(gamma1d1_50_0_opposite))) + px232_opposite +(beta1d1_50_left_up(1)-(beta1d1_50_0_opposite));

Ocline_x = px31_opposite*gamma+d3;
Odline_x = px41_opposite*gamma+d4;


if gamma < g4
    Obline_x = oobeta2_cal_1;
elseif gamma > g3
    Obline_x = oobeta2_cal_3;
else
    Obline_x = oobeta2_cal;
end

if gamma < g1
    Oaline_x = oobeta1_cal_1;
elseif gamma > g2
    Oaline_x = oobeta1_cal_3;
else
    Oaline_x = oobeta1_cal;
end
%% 内区域
gamma1dn_55=gamma1dn_50_left_down+1.9127;
beta1dn_55=beta1dn_50_left_down+0.0468;
gamma11_55=gamma11_50_right_down-0.0326;
beta11_55=beta11_50_right_down-0.1910;
gamma1d1_55=gamma1d1_50_left_up-0.0500;
beta1d1_55=beta1d1_50_left_up+0.1928;
gamma1n_55=gamma1n_50_right_up-1.8954;
beta1n_55=beta1n_50_right_up-0.0450;

px11 = -0.0297;
px12 = 0.1262;
px13 = -0.05774;
px21 = 0.5321 ;
px22 = -1.053;
px23 = 0.6621 ;
px24 = -0.2105 ;
px25 = 0.1441;
px26 = -0.03386 ;
px31 = 0.0297   ;
px32 = 0.1252   ;
px33 = 0.05739 ;
px41 =    0.5321;
px42 =    1.107 ;
px43 =    0.75;
px44 =    0.2536  ;
px45 =    0.1536  ;
px46 =   0.03542 ;
px51 = -0.06873  ;%(-21.16, -21.16)
px52 = 0.105;% (2.222, 2.222)
px61 = -0.06873  ;%(-21.16, -21.16)
px62 = -0.105 ;%(-2.222, -2.222)
d5=beta11_55-px51*gamma11_55;
d6=beta1d1_55-px61*gamma1d1_55;


Ibline_x = px21*(gamma-(gamma1d1_55(1)-(-0.213))).^5 + px22*(gamma-(gamma1d1_55(1)-(-0.213))).^4 + px23*(gamma-(gamma1d1_55(1)-(-0.213))).^3 + px24*(gamma-(gamma1d1_55(1)-(-0.213))).^2 + px25*(gamma-(gamma1d1_55(1)-(-0.213))) + px26+(beta1d1_55(1)-(-0.0860));
Ialine_x = px41*(gamma-(gamma1dn_55(1)-(-0.9591))).^5 + px42*(gamma-(gamma1dn_55(1)-(-0.9591))).^4 + px43*(gamma-(gamma1dn_55(1)-(-0.9591))).^3 + px44*(gamma-(gamma1dn_55(1)-(-0.9591))).^2 + px45*(gamma-(gamma1dn_55(1)-(-0.9591))) + px46+(beta1dn_55(1)-(-0.0354));
Icline_x = px51*gamma+d5;
Idline_x = px61*gamma+d6;   
   
%% 判断region
if beta <= min(Icline_x,Ialine_x) && beta >= max(Ibline_x,Idline_x)
    region=1;
elseif beta >= min(Ocline_x,Oaline_x) || beta <= max(Obline_x,Odline_x)
    region=3;
else
    region=2;
end

%% 得到index

left_Ix = max(Ibline_x,Idline_x);%k^{bd}_{in},phi1
right_Ix = min(Ialine_x,Icline_x);%k^{ac}_{in}
right_Ox = min(Oaline_x,Ocline_x);%k^{ac}_{out}
left_Ox = max(Obline_x,Odline_x);%k^{bd}_{out}

if region==1
    
    Center = (left_Ix + right_Ix)/2;
    if Center <= beta && beta <= right_Ix
        index = (right_Ix-beta)/right_Ix;
    else%if Center > beta && beta >= left_Ix
        index = (left_Ix-beta)/left_Ix;
    end
    
else%if region==2
    
    if beta >= right_Ix
        index = (-beta+right_Ix)/(right_Ox-right_Ix);
    else%if beta <= left_Ix
        index = (-beta+left_Ix)/(left_Ox-left_Ix);
    end
     
end
elseif Vx_kmh > 52.5 && Vx_kmh <= 57.5
   %% 外边界
for n=1:length(alpharl)
    if abs(alpharl(n))<abs(kekoalphaf)%%鐢ㄤ笉瓒宠浆鍚戞椂鍓嶅悗杞晶鍋忚鐨勫ぇ灏忓叧绯荤瓫閫夊悎閫傜殑
    beta1_right(n)=((sw_angle-kekoalphaf)*lr-lf*alpharl(n))/(lf+lr);
    gamma1_right(n)=((sw_angle-kekoalphaf+alpharl(n))*Vx)/(lf+lr);
    end
end

   beta11_55_right_down=beta1_right(1);
   gamma11_55_right_down=gamma1_right(1);
   beta1n_55_right_up=beta1_right(length(beta1_right));
   gamma1n_55_right_up=gamma1_right(length(gamma1_right));
   
    centerx_55=beta1n_55_right_up-0.0829;
    centery_55=gamma1n_55_right_up-3.1589;
   
    beta1d1_55_left_up=2*centerx_55-beta1_right(1);
    gamma1d1_55_left_up=2*centery_55-gamma1_right(1);
    beta1dn_55_left_down=2*centerx_55-beta1_right(length(beta1_right));
    gamma1dn_55_left_down=2*centery_55-gamma1_right(length(gamma1_right));
    
g1=2.3476+gamma1dn_55_left_down;
b1=0.0504+beta1dn_55_left_down;
g2=0.9743+g1;
b2=0.0993+b1;
g3=2*centery_55-g1;%%-g1
b3=2*centerx_55-b1;%%-b1
g4=2*centery_55-g2;%%-g2
b4=2*centerx_55-b2;%%-b2

%x11=gamma1dn_55_left_down:0.000005:g1;
       px111_opposite =     0.02147 ;
       px112_opposite =     -0.01509;
%x12=g1:0.000005:g2;
       px121_opposite =       0.5573 ;
       px122_opposite =        0.9644;
       px123_opposite =       0.5711 ;
       px124_opposite =       0.1918 ;
       px125_opposite =        0.1389  ;
       px126_opposite =      0.03643  ;
%x13=g2:0.000005:gamma11_55_right_down;
       px131_opposite =     1.692 ;% (-5.636e+05, -2.701e+05)
       px132_opposite =      -0.209;% (-6.956e+04, -3.484e+04)
%x21=gamma1d1_55_left_up:0.000005:g4;
       px211_opposite =        1.692 ;
       px212_opposite =        0.2089;
%x22= g4:0.000005:g3;
       px221_opposite =        0.5573;% (-6.388e+05, -3.304e+05)
       px222_opposite =       -0.9644;% (4.151e+04, 8.218e+04)
       px223_opposite =        0.5711 ;%  (-561.4, 843.6)
       px224_opposite =        -0.1918;% (-313, -264.4)
       px225_opposite =      0.1389 ;%  (18.8, 19.9)
       px226_opposite =     -0.03643 ;% (-0.3822, -0.3702)
%x23=g3:0.000005:gamma1n_55_right_up;
       px231_opposite =     0.02147 ;% (-5.636e+05, -2.701e+05)
       px232_opposite =      0.01508;% (-6.956e+04, -3.484e+04)
%x33=gamma11_55_right_down:0.000005:gamma1n_55_right_up;   
        px31_opposite =       -0.06873  ;%(-21.16, -21.16)
       px32_opposite =       0.3 ;% (2.222, 2.222)
%x44=gamma1dn_55_left_down:0.000005:gamma1d1_55_left_up; 
       px41_opposite =       -0.06873 ;%(-21.16, -21.16)
       px42_opposite =       -0.3 ;%(-2.222, -2.222)
d3=beta11_55_right_down-px31_opposite*gamma11_55_right_down;
d4=beta1d1_55_left_up-px41_opposite*gamma1d1_55_left_up;
gamma1dn_55_0_opposite= -3.1589;
beta1dn_55_0_opposite=-0.0829;
gamma1d1_55_0_opposite=-0.2891;
beta1d1_55_0_opposite=-0.2801;     
       
oobeta1_cal_1 = px111_opposite*(gamma-(gamma1dn_55_left_down(1)-(gamma1dn_55_0_opposite))) + px112_opposite +(beta1dn_55_left_down(1)-(beta1dn_55_0_opposite));
oobeta1_cal = px121_opposite*(gamma-(gamma1dn_55_left_down(1)-(gamma1dn_55_0_opposite))).^5 + px122_opposite*(gamma-(gamma1dn_55_left_down(1)-(gamma1dn_55_0_opposite))).^4 + px123_opposite*(gamma-(gamma1dn_55_left_down(1)-(gamma1dn_55_0_opposite))).^3 + px124_opposite*(gamma-(gamma1dn_55_left_down(1)-(gamma1dn_55_0_opposite))).^2 + px125_opposite*(gamma-(gamma1dn_55_left_down(1)-(gamma1dn_55_0_opposite))) + px126_opposite+(beta1dn_55_left_down(1)-(beta1dn_55_0_opposite));
oobeta1_cal_3 = px131_opposite*(gamma-(gamma1dn_55_left_down(1)-(gamma1dn_55_0_opposite))) + px132_opposite +(beta1dn_55_left_down(1)-(beta1dn_55_0_opposite));
oobeta2_cal_1 = px211_opposite*(gamma-(gamma1d1_55_left_up(1)-(gamma1d1_55_0_opposite))) + px212_opposite +(beta1d1_55_left_up(1)-(beta1d1_55_0_opposite));
oobeta2_cal = px221_opposite*(gamma-(gamma1d1_55_left_up(1)-(gamma1d1_55_0_opposite))).^5 + px222_opposite*(gamma-(gamma1d1_55_left_up(1)-(gamma1d1_55_0_opposite))).^4 + px223_opposite*(gamma-(gamma1d1_55_left_up(1)-(gamma1d1_55_0_opposite))).^3 + px224_opposite*(gamma-(gamma1d1_55_left_up(1)-(gamma1d1_55_0_opposite))).^2 + px225_opposite*(gamma-(gamma1d1_55_left_up(1)-(gamma1d1_55_0_opposite))) + px226_opposite+(beta1d1_55_left_up(1)-(beta1d1_55_0_opposite));
oobeta2_cal_3 = px231_opposite*(gamma-(gamma1d1_55_left_up(1)-(gamma1d1_55_0_opposite))) + px232_opposite +(beta1d1_55_left_up(1)-(beta1d1_55_0_opposite));

Ocline_x = px31_opposite*gamma+d3;
Odline_x = px41_opposite*gamma+d4;


if gamma < g4
    Obline_x = oobeta2_cal_1;
elseif gamma > g3
    Obline_x = oobeta2_cal_3;
else
    Obline_x = oobeta2_cal;
end

if gamma < g1
    Oaline_x = oobeta1_cal_1;
elseif gamma > g2
    Oaline_x = oobeta1_cal_3;
else
    Oaline_x = oobeta1_cal;
end
%% 内边界
gamma1dn_60=gamma1dn_55_left_down+2.0937;
beta1dn_60=beta1dn_55_left_down+0.0450;
gamma11_60=gamma11_55_right_down-0.0380;
beta11_60=beta11_55_right_down-0.1910;
gamma1d1_60=gamma1d1_55_left_up+0.0379;
beta1d1_60=beta1d1_55_left_up+0.1910;
gamma1n_60=gamma1n_55_right_up -2.0938;
beta1n_60=beta1n_55_right_up-0.0450;

px11 =     -0.02516   ;
px12 =      0.1158;
px13 =      -0.05754 ;
px21 =       0.2115 ;
px22 =       -0.4953 ;
px23 =       0.4081 ;
px24 =        -0.2025 ;
px25 =      0.1451;
px26 =    -0.0325 ;
px31 =       0.02516   ;
px32 =       0.1158   ;
px33 =       0.05754 ;
px41 =    0.2115;
px42 =    0.477 ;
px43 =    0.3744;
px44 =    0.1822  ;
px45 =    0.1384   ;
px46 =    0.03188 ;
px51 =     -0.063 ;%(-21.16, -21.16)
px52 =      0.105 ;% (2.222, 2.222)
px61 =    -0.063  ;%(-21.16, -21.16)
px62 =    -0.105 ;%(-2.222, -2.222)
d5=beta11_60-px51*gamma11_60;
d6=beta1d1_60-px61*gamma1d1_60;

Ibline_x = px21*(gamma-(gamma1d1_60(1)-(-0.2512))).^5 + px22*(gamma-(gamma1d1_60(1)-(-0.2512))).^4 + px23*(gamma-(gamma1d1_60(1)-(-0.2512))).^3 + px24*(gamma-(gamma1d1_60(1)-(-0.2512))).^2 + px25*(gamma-(gamma1d1_60(1)-(-0.2512))) + px26+(beta1d1_60(1)-(-0.0882));
Ialine_x = px41*(gamma-(gamma1dn_60(1)-(-1.0652))).^5 + px42*(gamma-(gamma1dn_60(1)-(-1.0652))).^4 + px43*(gamma-(gamma1dn_60(1)-(-1.0652))).^3 + px44*(gamma-(gamma1dn_60(1)-(-1.0652))).^2 + px45*(gamma-(gamma1dn_60(1)-(-1.0652))) + px46+(beta1dn_60(1)-( -0.0373));
Icline_x = px51*gamma+d5;
Idline_x = px61*gamma+d6;

%% 判断region
if beta <= min(Icline_x,Ialine_x) && beta >= max(Ibline_x,Idline_x)
    region=1;
elseif beta >= min(Ocline_x,Oaline_x) || beta <= max(Obline_x,Odline_x)
    region=3;
else
    region=2;
end

%% 得到index

left_Ix = max(Ibline_x,Idline_x);%k^{bd}_{in},phi1
right_Ix = min(Ialine_x,Icline_x);%k^{ac}_{in}
right_Ox = min(Oaline_x,Ocline_x);%k^{ac}_{out}
left_Ox = max(Obline_x,Odline_x);%k^{bd}_{out}

if region==1
    
    Center = (left_Ix + right_Ix)/2;
    if Center <= beta && beta <= right_Ix
        index = (right_Ix-beta)/right_Ix;
    else%if Center > beta && beta >= left_Ix
        index = (left_Ix-beta)/left_Ix;
    end
    
else%if region==2
    
    if beta >= right_Ix
        index = (-beta+right_Ix)/(right_Ox-right_Ix);
    else%if beta <= left_Ix
        index = (-beta+left_Ix)/(left_Ox-left_Ix);
    end
     
end
elseif Vx_kmh >= 57.5 && Vx_kmh <= 62.5  %60
    %% 外边界
for n=1:length(alpharl)
    if abs(alpharl(n))<abs(kekoalphaf)%%鐢ㄤ笉瓒宠浆鍚戞椂鍓嶅悗杞晶鍋忚鐨勫ぇ灏忓叧绯荤瓫閫夊悎閫傜殑
    beta1_right(n)=((sw_angle-kekoalphaf)*lr-lf*alpharl(n))/(lf+lr);
    gamma1_right(n)=((sw_angle-kekoalphaf+alpharl(n))*Vx)/(lf+lr);
    end
end

   beta11_60_right_down=beta1_right(1);
   gamma11_60_right_down=gamma1_right(1);
   beta1n_60_right_up=beta1_right(length(beta1_right));
   gamma1n_60_right_up=gamma1_right(length(gamma1_right));
   
    centerx_60=beta1n_60_right_up-0.0829;
    centery_60=gamma1n_60_right_up-3.4461;
   
    beta1d1_60_left_up=2*centerx_60-beta1_right(1);
    gamma1d1_60_left_up=2*centery_60-gamma1_right(1);
    beta1dn_60_left_down=2*centerx_60-beta1_right(length(beta1_right));
    gamma1dn_60_left_down=2*centery_60-gamma1_right(length(gamma1_right));
    
g1=2.5611+gamma1dn_60_left_down;
b1=0.0504+beta1dn_60_left_down;
g2=1.0628+g1;
b2=0.0993+b1;
g3=2*centery_60-g1;%%-g1
b3=2*centerx_60-b1;%%-b1
g4=2*centery_60-g2;%%-g2
b4=2*centerx_60-b2;%%-b2

%x11=gamma1dn_60_left_down:0.000005:g1;
       px111_opposite =      0.01968 ;
       px112_opposite =      -0.01509;
%x12=g1:0.000005:g2;
       px121_opposite =        0.2999 ;
       px122_opposite =        0.5752;
       px123_opposite =        0.4018;
       px124_opposite =       0.1778;
       px125_opposite =       0.1346 ;
       px126_opposite =       0.03535;
%x13=g2:0.000005:gamma11_60_right_down;
       px131_opposite =     1.55;% (-5.636e+05, -2.701e+05)
       px132_opposite =    -0.2089;% (-6.956e+04, -3.484e+04)
% x21=gamma1d1_60_left_up:0.000005:g4;
       px211_opposite =        1.55 ;
       px212_opposite =         0.2088;
% x22= g4:0.000005:g3;
       px221_opposite =         0.2999;% (-6.388e+05, -3.304e+05)
       px222_opposite =        -0.5752;% (4.151e+04, 8.218e+04)
       px223_opposite =          0.4018 ;%  (-561.4, 843.6)
       px224_opposite =       -0.1778 ;% (-313, -264.4)
       px225_opposite =       0.1346  ;%  (18.8, 19.9)
       px226_opposite =      -0.03535 ;% (-0.3822, -0.3702)
% x23=g3:0.000005:gamma1n_60_right_up;
       px231_opposite =    0.01968 ;% (-5.636e+05, -2.701e+05)
       px232_opposite =       0.01508;% (-6.956e+04, -3.484e+04)
% x33=gamma11_60_right_down:0.000005:gamma1n_60_right_up;   
       px31_opposite =       -0.063 ;%(-21.16, -21.16)
       px32_opposite =       0.3 ;% (2.222, 2.222)
% x44=gamma1dn_60_left_down:0.000005:gamma1d1_60_left_up; 
       px41_opposite =      -0.063 ;%(-21.16, -21.16)
       px42_opposite =       -0.3 ;%(-2.222, -2.222)
d3=beta11_60_right_down-px31_opposite*gamma11_60_right_down;
d4=beta1d1_60_left_up-px41_opposite*gamma1d1_60_left_up;
gamma1dn_60_0_opposite= -3.4461;
beta1dn_60_0_opposite=-0.0829;
gamma1d1_60_0_opposite=-0.3154;
beta1d1_60_0_opposite=-0.2801;  
       
oobeta1_cal_1 = px111_opposite*(gamma-(gamma1dn_60_left_down(1)-(gamma1dn_60_0_opposite))) + px112_opposite +(beta1dn_60_left_down(1)-(beta1dn_60_0_opposite));
oobeta1_cal = px121_opposite*(gamma-(gamma1dn_60_left_down(1)-(gamma1dn_60_0_opposite))).^5 + px122_opposite*(gamma-(gamma1dn_60_left_down(1)-(gamma1dn_60_0_opposite))).^4 + px123_opposite*(gamma-(gamma1dn_60_left_down(1)-(gamma1dn_60_0_opposite))).^3 + px124_opposite*(gamma-(gamma1dn_60_left_down(1)-(gamma1dn_60_0_opposite))).^2 + px125_opposite*(gamma-(gamma1dn_60_left_down(1)-(gamma1dn_60_0_opposite))) + px126_opposite+(beta1dn_60_left_down(1)-(beta1dn_60_0_opposite));
oobeta1_cal_3 = px131_opposite*(gamma-(gamma1dn_60_left_down(1)-(gamma1dn_60_0_opposite))) + px132_opposite +(beta1dn_60_left_down(1)-(beta1dn_60_0_opposite));
oobeta2_cal_1 = px211_opposite*(gamma-(gamma1d1_60_left_up(1)-(gamma1d1_60_0_opposite))) + px212_opposite +(beta1d1_60_left_up(1)-(beta1d1_60_0_opposite));
oobeta2_cal = px221_opposite*(gamma-(gamma1d1_60_left_up(1)-(gamma1d1_60_0_opposite))).^5 + px222_opposite*(gamma-(gamma1d1_60_left_up(1)-(gamma1d1_60_0_opposite))).^4 + px223_opposite*(gamma-(gamma1d1_60_left_up(1)-(gamma1d1_60_0_opposite))).^3 + px224_opposite*(gamma-(gamma1d1_60_left_up(1)-(gamma1d1_60_0_opposite))).^2 + px225_opposite*(gamma-(gamma1d1_60_left_up(1)-(gamma1d1_60_0_opposite))) + px226_opposite+(beta1d1_60_left_up(1)-(beta1d1_60_0_opposite));
oobeta2_cal_3 = px231_opposite*(gamma-(gamma1d1_60_left_up(1)-(gamma1d1_60_0_opposite))) + px232_opposite +(beta1d1_60_left_up(1)-(beta1d1_60_0_opposite));


Ocline_x = px31_opposite*gamma+d3;
Odline_x = px41_opposite*gamma+d4;


if gamma < g4
    Obline_x = oobeta2_cal_1;
elseif gamma > g3
    Obline_x = oobeta2_cal_3;
else
    Obline_x = oobeta2_cal;
end

if gamma < g1
    Oaline_x = oobeta1_cal_1;
elseif gamma > g2
    Oaline_x = oobeta1_cal_3;
else
    Oaline_x = oobeta1_cal;
end
%% 内边界
gamma1dn_65=gamma1dn_60_left_down+2.3126;
beta1dn_65=beta1dn_60_left_down+0.0468;
gamma11_65=gamma11_60_right_down-0.0433;
beta11_65=beta11_60_right_down-0.1910;
gamma1d1_65=gamma1d1_60_left_up+0.0637;
beta1d1_65=beta1d1_60_left_up+0.1928;
gamma1n_65=gamma1n_60_right_up-2.2922;
beta1n_65=beta1n_60_right_up-0.0450;

px11 =    -0.02209    ;
px12 =      0.1075 ;
px13 =     -0.05744 ;
px21 =     -0.03903 ;
px22 =      0.02466 ;
px23 =      0.1071 ;
px24 =     -0.1725 ;
px25 =      0.1474;
px26 =   -0.03098 ;
px31 =      0.02209  ;
px32 =       0.1066 ;
px33 =       0.05707 ;
px41 =    -0.03903;
px42 =   -0.02466 ;
px43 =    0.1071 ;
px44 =     0.1725  ;
px45 =    0.1474  ;
px46 =   0.03098 ;
px51 =      -0.05815   ;%(-21.16, -21.16)
px52 =        0.105 ;% (2.222, 2.222)
px61 =    -0.05815  ;%(-21.16, -21.16)
px62 =    -0.105 ;%(-2.222, -2.222)
d5=beta11_65-px51*gamma11_65;
d6=beta1d1_65-px61*gamma1d1_65;

Ibline_x = px21*(gamma-(gamma1d1_65(1)-(-0.2517))).^5 + px22*(gamma-(gamma1d1_65(1)-(-0.2517))).^4 + px23*(gamma-(gamma1d1_65(1)-(-0.2517))).^3 + px24*(gamma-(gamma1d1_65(1)-(-0.2517))).^2 + px25*(gamma-(gamma1d1_65(1)-(-0.2517))) + px26+(beta1d1_65(1)-(-0.0859));
Ialine_x = px41*(gamma-(gamma1dn_65(1)-(-1.1335))).^5 + px42*(gamma-(gamma1dn_65(1)-(-1.1335))).^4 + px43*(gamma-(gamma1dn_65(1)-(-1.1335))).^3 + px44*(gamma-(gamma1dn_65(1)-(-1.1335))).^2 + px45*(gamma-(gamma1dn_65(1)-(-1.1335))) + px46+(beta1dn_65(1)-(-0.0354));
Icline_x = px51*gamma+d5;
Idline_x = px61*gamma+d6;

%% 判断region
if beta <= min(Icline_x,Ialine_x) && beta >= max(Ibline_x,Idline_x)
    region=1;
elseif beta >= min(Ocline_x,Oaline_x) || beta <= max(Obline_x,Odline_x)
    region=3;
else
    region=2;
end

%% 得到index

left_Ix = max(Ibline_x,Idline_x);%k^{bd}_{in},phi1
right_Ix = min(Ialine_x,Icline_x);%k^{ac}_{in}
right_Ox = min(Oaline_x,Ocline_x);%k^{ac}_{out}
left_Ox = max(Obline_x,Odline_x);%k^{bd}_{out}

if region==1
    
    Center = (left_Ix + right_Ix)/2;
    if Center <= beta && beta <= right_Ix
        index = (right_Ix-beta)/right_Ix;
    else%if Center > beta && beta >= left_Ix
        index = (left_Ix-beta)/left_Ix;
    end
    
else%if region==2
    
    if beta >= right_Ix
        index = (-beta+right_Ix)/(right_Ox-right_Ix);
    else%if beta <= left_Ix
        index = (-beta+left_Ix)/(left_Ox-left_Ix);
    end
     
end
elseif Vx_kmh > 62.5 && Vx_kmh<=67.5%65
    %% 外边界
for n=1:length(alpharl)
    if abs(alpharl(n))<abs(kekoalphaf)%%鐢ㄤ笉瓒宠浆鍚戞椂鍓嶅悗杞晶鍋忚鐨勫ぇ灏忓叧绯荤瓫閫夊悎閫傜殑
    beta1_right(n)=((sw_angle-kekoalphaf)*lr-lf*alpharl(n))/(lf+lr);
    gamma1_right(n)=((sw_angle-kekoalphaf+alpharl(n))*Vx)/(lf+lr);
    end
end

   beta11_65_right_down=beta1_right(1);
   gamma11_65_right_down=gamma1_right(1);
   beta1n_65_right_up=beta1_right(length(beta1_right));
   gamma1n_65_right_up=gamma1_right(length(gamma1_right));
   
   centerx_65=beta1n_65_right_up-0.0829;
    centery_65=gamma1n_65_right_up-3.7333;
   
  beta1d1_65_left_up=2*centerx_65-beta1_right(1);%鍒╃敤涓偣鍏紡姹傚绉扮偣
    gamma1d1_65_left_up=2*centery_65-gamma1_right(1);%鍒╃敤涓偣鍏紡姹傚绉扮偣
    beta1dn_65_left_down=2*centerx_65-beta1_right(length(beta1_right));%鍒╃敤涓偣鍏紡姹傚绉扮偣
    gamma1dn_65_left_down=2*centery_65-gamma1_right(length(gamma1_right));%鍒╃敤涓偣鍏紡姹傚绉扮偣
    
g1=2.9069+gamma1dn_65_left_down;
b1=0.0571+beta1dn_65_left_down;
g2= 1.0028+g1;
b2=  0.0894+b1;
g3=2*centery_65-g1;%%-g1
b3=2*centerx_65-b1;%%-b1
g4=2*centery_65-g2;%%-g2
b4=2*centerx_65-b2;%%-b2


% x11=gamma1dn_65_left_down:0.000005:g1;
       px111_opposite =      0.01964;
       px112_opposite =     -0.009572;
% x12=g1:0.000005:g2;
       px121_opposite =        0.1566   ;
       px122_opposite =        0.3053;
       px123_opposite =        0.2651;
       px124_opposite =        0.1741;
       px125_opposite =        0.1348  ;
       px126_opposite =       0.03383;
% x13=g2:0.000005:gamma11_65_right_down;
       px131_opposite =    1.31;% (-5.636e+05, -2.701e+05)
       px132_opposite =     -0.1674;% (-6.956e+04, -3.484e+04)
% x21=gamma1d1_65_left_up:0.000005:g4;
       px211_opposite =       1.31 ;
       px212_opposite =          0.1675;
% x22= g4:0.000005:g3;
       px221_opposite =         0.1566 ;% (-6.388e+05, -3.304e+05)
       px222_opposite =         -0.3053;% (4.151e+04, 8.218e+04)
       px223_opposite =          0.2651  ;%  (-561.4, 843.6)
       px224_opposite =        -0.1741 ;% (-313, -264.4)
       px225_opposite =          0.1348;%  (18.8, 19.9)
       px226_opposite =       -0.03383;% (-0.3822, -0.3702)
% x23=g3:0.000005:gamma1n_65_right_up;
       px231_opposite =     0.01964;% (-5.636e+05, -2.701e+05)
       px232_opposite =        0.009562;% (-6.956e+04, -3.484e+04)
% x33=gamma11_65_right_down:0.000005:gamma1n_65_right_up;   
       px31_opposite =       -0.05815 ;%(-21.16, -21.16)
       px32_opposite =       0.3 ;% (2.222, 2.222)
% x44=gamma1dn_65_left_down:0.000005:gamma1d1_65_left_up; 
       px41_opposite =     -0.05815;%(-21.16, -21.16)
       px42_opposite =       -0.3 ;%(-2.222, -2.222)
d3=beta11_65_right_down-px31_opposite*gamma11_65_right_down;
d4=beta1d1_65_left_up-px41_opposite*gamma1d1_65_left_up;
gamma1dn_65_0_opposite= -3.7333;
beta1dn_65_0_opposite=-0.0829;
gamma1d1_65_0_opposite=-0.3417;
beta1d1_65_0_opposite=-0.2801;
       
oobeta1_cal_1 = px111_opposite*(gamma-(gamma1dn_65_left_down(1)-(gamma1dn_65_0_opposite))) + px112_opposite +(beta1dn_65_left_down(1)-(beta1dn_65_0_opposite));
oobeta1_cal = px121_opposite*(gamma-(gamma1dn_65_left_down(1)-(gamma1dn_65_0_opposite))).^5 + px122_opposite*(gamma-(gamma1dn_65_left_down(1)-(gamma1dn_65_0_opposite))).^4 + px123_opposite*(gamma-(gamma1dn_65_left_down(1)-(gamma1dn_65_0_opposite))).^3 + px124_opposite*(gamma-(gamma1dn_65_left_down(1)-(gamma1dn_65_0_opposite))).^2 + px125_opposite*(gamma-(gamma1dn_65_left_down(1)-(gamma1dn_65_0_opposite))) + px126_opposite+(beta1dn_65_left_down(1)-(beta1dn_65_0_opposite));
oobeta1_cal_3 = px131_opposite*(gamma-(gamma1dn_65_left_down(1)-(gamma1dn_65_0_opposite))) + px132_opposite +(beta1dn_65_left_down(1)-(beta1dn_65_0_opposite));
oobeta2_cal_1 = px211_opposite*(gamma-(gamma1d1_65_left_up(1)-(gamma1d1_65_0_opposite))) + px212_opposite +(beta1d1_65_left_up(1)-(beta1d1_65_0_opposite));
oobeta2_cal = px221_opposite*(gamma-(gamma1d1_65_left_up(1)-(gamma1d1_65_0_opposite))).^5 + px222_opposite*(gamma-(gamma1d1_65_left_up(1)-(gamma1d1_65_0_opposite))).^4 + px223_opposite*(gamma-(gamma1d1_65_left_up(1)-(gamma1d1_65_0_opposite))).^3 + px224_opposite*(gamma-(gamma1d1_65_left_up(1)-(gamma1d1_65_0_opposite))).^2 + px225_opposite*(gamma-(gamma1d1_65_left_up(1)-(gamma1d1_65_0_opposite))) + px226_opposite+(beta1d1_65_left_up(1)-(beta1d1_65_0_opposite));
oobeta2_cal_3 = px231_opposite*(gamma-(gamma1d1_65_left_up(1)-(gamma1d1_65_0_opposite))) + px232_opposite +(beta1d1_65_left_up(1)-(beta1d1_65_0_opposite));

Ocline_x = px31_opposite*gamma+d3;
Odline_x = px41_opposite*gamma+d4;

if gamma < g4
    Obline_x = oobeta2_cal_1;
elseif gamma > g3
    Obline_x = oobeta2_cal_3;
else
    Obline_x = oobeta2_cal;
end

if gamma < g1
    Oaline_x = oobeta1_cal_1;
elseif gamma > g2
    Oaline_x = oobeta1_cal_3;
else
    Oaline_x = oobeta1_cal;
end
%% 内边界
gamma1dn_70=gamma1dn_65_left_down+2.4906;
beta1dn_70=beta1dn_65_left_down+0.0450;
gamma11_70=gamma11_65_right_down-0.0487;
beta11_70=beta11_65_right_down-0.1910;
gamma1d1_70=gamma1d1_65_left_up+0.0487;
beta1d1_70=beta1d1_65_left_up+0.1910;
gamma1n_70=gamma1n_65_right_up-2.4906;
beta1n_70=beta1n_65_right_up-0.0450;

px11 =     -0.01907    ;
px12 =      0.09987;
px13 =      -0.05743 ;
px21 =       -0.03646;
px22 =       0.02589;
px23 =       0.1129 ;
px24 =       -0.1822 ;
px25 =     0.1435;
px26 =    -0.02931 ;
px31 =      0.01907   ;
px32 =       0.09987   ;
px33 =       0.05743  ;
px41 =    -0.03646;
px42 =    -0.02217 ;
px43 =    0.1148;
px44 =    0.1752 ;
px45 =    0.1362  ;
px46 =   0.02828 ;
px51 =     -0.054  ;%(-21.16, -21.16)
px52 =      0.105 ;% (2.222, 2.222)
px61 =    -0.054 ;%(-21.16, -21.16)
px62 =    -0.105 ;%(-2.222, -2.222)
d5=beta11_70-px51*gamma11_70;
d6=beta1d1_70-px61*gamma1d1_70;

Ibline_x = px21*(gamma-(gamma1d1_70(1)-(-0.2930))).^5 + px22*(gamma-(gamma1d1_70(1)-(-0.2930))).^4 + px23*(gamma-(gamma1d1_70(1)-(-0.2930))).^3 + px24*(gamma-(gamma1d1_70(1)-(-0.2930))).^2 + px25*(gamma-(gamma1d1_70(1)-(-0.2930))) + px26+(beta1d1_70(1)-( -0.0883));
Ialine_x = px41*(gamma-(gamma1dn_70(1)-(-1.2427))).^5 + px42*(gamma-(gamma1dn_70(1)-(-1.2427))).^4 + px43*(gamma-(gamma1dn_70(1)-(-1.2427))).^3 + px44*(gamma-(gamma1dn_70(1)-(-1.2427))).^2 + px45*(gamma-(gamma1dn_70(1)-(-1.2427))) + px46+(beta1dn_70(1)-(-0.0372));
Icline_x = px51*gamma+d5;
Idline_x = px61*gamma+d6;   
%% 判断region
if beta <= min(Icline_x,Ialine_x) && beta >= max(Ibline_x,Idline_x)
    region=1;
elseif beta >= min(Ocline_x,Oaline_x) || beta <= max(Obline_x,Odline_x)
    region=3;
else
    region=2;
end

%% 得到index

left_Ix = max(Ibline_x,Idline_x);%k^{bd}_{in},phi1
right_Ix = min(Ialine_x,Icline_x);%k^{ac}_{in}
right_Ox = min(Oaline_x,Ocline_x);%k^{ac}_{out}
left_Ox = max(Obline_x,Odline_x);%k^{bd}_{out}

if region==1
    
    Center = (left_Ix + right_Ix)/2;
    if Center <= beta && beta <= right_Ix
        index = (right_Ix-beta)/right_Ix;
    else%if Center > beta && beta >= left_Ix
        index = (left_Ix-beta)/left_Ix;
    end
    
else%if region==2
    
    if beta >= right_Ix
        index = (-beta+right_Ix)/(right_Ox-right_Ix);
    else%if beta <= left_Ix
        index = (-beta+left_Ix)/(left_Ox-left_Ix);
    end
     
end
elseif Vx_kmh > 67.5 && Vx_kmh <= 72.5%70
    %% 外边界
for n=1:length(alpharl)
    if abs(alpharl(n))<abs(kekoalphaf)%%鐢ㄤ笉瓒宠浆鍚戞椂鍓嶅悗杞晶鍋忚鐨勫ぇ灏忓叧绯荤瓫閫夊悎閫傜殑
    beta1_right(n)=((sw_angle-kekoalphaf)*lr-lf*alpharl(n))/(lf+lr);
    gamma1_right(n)=((sw_angle-kekoalphaf+alpharl(n))*Vx)/(lf+lr);
    end
end

   beta11_70_right_down=beta1_right(1);
   gamma11_70_right_down=gamma1_right(1);
   beta1n_70_right_up=beta1_right(length(beta1_right));
   gamma1n_70_right_up=gamma1_right(length(gamma1_right));
   
   centerx_70=beta1n_70_right_up-0.0829;
    centery_70=gamma1n_70_right_up-4.0205;
   
    beta1d1_70_left_up=2*centerx_70-beta1_right(1);%鍒╃敤涓偣鍏紡姹傚绉扮偣
    gamma1d1_70_left_up=2*centery_70-gamma1_right(1);%鍒╃敤涓偣鍏紡姹傚绉扮偣
    beta1dn_70_left_down=2*centerx_70-beta1_right(length(beta1_right));%鍒╃敤涓偣鍏紡姹傚绉扮偣
    gamma1dn_70_left_down=2*centery_70-gamma1_right(length(gamma1_right));%鍒╃敤涓偣鍏紡姹傚绉扮偣
    
g1=3.1305+gamma1dn_70_left_down;%璁＄畻ogamma2_down(1)-gamma1dn_70_left_down=锛熶綔涓哄墠闈㈢殑涓�釜鍔犳暟;
b1=0.0571+beta1dn_70_left_down;%obeta2_down(1)-beta1dn_70_left_down=锛�
g2=1.0800+g1;%ogamma2_down(length(ogamma2_down))-ogamma2_down(1)=锛�
b2=0.0894+b1;%obeta2_down(length(obeta2_down))-obeta2_down(1)=锛�
g3=2*centery_70-g1;%%-g1
b3=2*centerx_70-b1;%%-b1
g4=2*centery_70-g2;%%-g2
b4=2*centerx_70-b2;%%-b2


% x11=gamma1dn_70_left_down:0.000005:g1;
       px111_opposite =       0.01824;
       px112_opposite =      -0.009571;
% x12=g1:0.000005:g2;
       px121_opposite =        -0.1022   ;
       px122_opposite =         -0.1346;
       px123_opposite =         0.05351;
       px124_opposite =         0.1623;
       px125_opposite =         0.137 ;
       px126_opposite =       0.03278;
% x13=g2:0.000005:gamma11_70_right_down;
       px131_opposite =   1.216;% (-5.636e+05, -2.701e+05)
       px132_opposite =    -0.1675;% (-6.956e+04, -3.484e+04)
% x21=gamma1d1_70_left_up:0.000005:g4;
       px211_opposite =       1.216 ;
       px212_opposite =       0.1675;
% x22= g4:0.000005:g3;
       px221_opposite =       -0.1022  ;% (-6.388e+05, -3.304e+05)
       px222_opposite =         0.1346 ;% (4.151e+04, 8.218e+04)
       px223_opposite =        0.05351  ;%  (-561.4, 843.6)
       px224_opposite =         -0.1623 ;% (-313, -264.4)
       px225_opposite =           0.137;%  (18.8, 19.9)
       px226_opposite =        -0.03278;% (-0.3822, -0.3702)
% x23=g3:0.000005:gamma1n_70_right_up;
       px231_opposite =     0.01824;% (-5.636e+05, -2.701e+05)
       px232_opposite =      0.009562;% (-6.956e+04, -3.484e+04)
% x33=gamma11_70_right_down:0.000005:gamma1n_70_right_up;   
       px31_opposite =      -0.054;%(-21.16, -21.16)
       px32_opposite =       0.3 ;% (2.222, 2.222)
% x44=gamma1dn_70_left_down:0.000005:gamma1d1_70_left_up; 
       px41_opposite =     -0.054;%(-21.16, -21.16)
       px42_opposite =       -0.3 ;%(-2.222, -2.222)
d3=beta11_70_right_down-px31_opposite*gamma11_70_right_down;
d4=beta1d1_70_left_up-px41_opposite*gamma1d1_70_left_up;
gamma1dn_70_0_opposite= -4.0205;
beta1dn_70_0_opposite=-0.0829;
gamma1d1_70_0_opposite=-0.3681;
beta1d1_70_0_opposite=-0.2801;
       
oobeta1_cal_1 = px111_opposite*(gamma-(gamma1dn_70_left_down(1)-(gamma1dn_70_0_opposite))) + px112_opposite +(beta1dn_70_left_down(1)-(beta1dn_70_0_opposite));
oobeta1_cal = px121_opposite*(gamma-(gamma1dn_70_left_down(1)-(gamma1dn_70_0_opposite))).^5 + px122_opposite*(gamma-(gamma1dn_70_left_down(1)-(gamma1dn_70_0_opposite))).^4 + px123_opposite*(gamma-(gamma1dn_70_left_down(1)-(gamma1dn_70_0_opposite))).^3 + px124_opposite*(gamma-(gamma1dn_70_left_down(1)-(gamma1dn_70_0_opposite))).^2 + px125_opposite*(gamma-(gamma1dn_70_left_down(1)-(gamma1dn_70_0_opposite))) + px126_opposite+(beta1dn_70_left_down(1)-(beta1dn_70_0_opposite));
oobeta1_cal_3 = px131_opposite*(gamma-(gamma1dn_70_left_down(1)-(gamma1dn_70_0_opposite))) + px132_opposite +(beta1dn_70_left_down(1)-(beta1dn_70_0_opposite));
oobeta2_cal_1 = px211_opposite*(gamma-(gamma1d1_70_left_up(1)-(gamma1d1_70_0_opposite))) + px212_opposite +(beta1d1_70_left_up(1)-(beta1d1_70_0_opposite));
oobeta2_cal = px221_opposite*(gamma-(gamma1d1_70_left_up(1)-(gamma1d1_70_0_opposite))).^5 + px222_opposite*(gamma-(gamma1d1_70_left_up(1)-(gamma1d1_70_0_opposite))).^4 + px223_opposite*(gamma-(gamma1d1_70_left_up(1)-(gamma1d1_70_0_opposite))).^3 + px224_opposite*(gamma-(gamma1d1_70_left_up(1)-(gamma1d1_70_0_opposite))).^2 + px225_opposite*(gamma-(gamma1d1_70_left_up(1)-(gamma1d1_70_0_opposite))) + px226_opposite+(beta1d1_70_left_up(1)-(beta1d1_70_0_opposite));
oobeta2_cal_3 = px231_opposite*(gamma-(gamma1d1_70_left_up(1)-(gamma1d1_70_0_opposite))) + px232_opposite +(beta1d1_70_left_up(1)-(beta1d1_70_0_opposite));

Ocline_x = px31_opposite*gamma+d3;
Odline_x = px41_opposite*gamma+d4;

if gamma < g4
    Obline_x = oobeta2_cal_1;
elseif gamma > g3
    Obline_x = oobeta2_cal_3;
else
    Obline_x = oobeta2_cal;
end

if gamma < g1
    Oaline_x = oobeta1_cal_1;
elseif gamma > g2
    Oaline_x = oobeta1_cal_3;
else
    Oaline_x = oobeta1_cal;
end
%% 内边界
gamma1dn_75=gamma1dn_70_left_down+2.6891;
beta1dn_75=beta1dn_70_left_down+0.0450;
gamma11_75=gamma11_70_right_down-0.0540;
beta11_75=beta11_70_right_down-0.1910;
gamma1d1_75=gamma1d1_70_left_up+0.0541;
beta1d1_75=beta1d1_70_left_up+0.1910;
gamma1n_75=gamma1n_70_right_up-2.6890;
beta1n_75=beta1n_70_right_up-0.0450;

px11 =     -0.01691    ;
px12 =      0.09367 ;
px13 =     -0.05735 ;
px21 =      -0.06546 ;
px22 =       0.1056;
px23 =       0.05459  ;
px24 =       -0.1731 ;
px25 =      0.1397;
px26 =    -0.028 ;
px31 =       0.01691  ;
px32 =       0.09367  ;
px33 =        0.05735;
px41 =    -0.06546;
px42 =     -0.1056;
px43 =    0.05459;
px44 =    0.1731  ;
px45 =    0.1397  ;
px46 =   0.028 ;
px51 =     -0.0504  ;%(-21.16, -21.16)
px52 =      0.105;% (2.222, 2.222)
px61 =    -0.0504  ;%(-21.16, -21.16)
px62 =    -0.105 ;%(-2.222, -2.222)
d5=beta11_75-px51*gamma11_75;
d6=beta1d1_75-px61*gamma1d1_75;

Ibline_x = px21*(gamma-(gamma1d1_75(1)-(-0.3140))).^5 + px22*(gamma-(gamma1d1_75(1)-(-0.3140))).^4 + px23*(gamma-(gamma1d1_75(1)-(-0.3140))).^3 + px24*(gamma-(gamma1d1_75(1)-(-0.3140))).^2 + px25*(gamma-(gamma1d1_75(1)-(-0.3140))) + px26+(beta1d1_75(1)-(-0.0884));
Ialine_x = px41*(gamma-(gamma1dn_75(1)-(-1.3315))).^5 + px42*(gamma-(gamma1dn_75(1)-(-1.3315))).^4 + px43*(gamma-(gamma1dn_75(1)-(-1.3315))).^3 + px44*(gamma-(gamma1dn_75(1)-(-1.3315))).^2 + px45*(gamma-(gamma1dn_75(1)-(-1.3315))) + px46+(beta1dn_75(1)-(-0.0374));
Icline_x = px51*gamma+d5;
Idline_x = px61*gamma+d6;  
%% 判断region
if beta <= min(Icline_x,Ialine_x) && beta >= max(Ibline_x,Idline_x)
    region=1;
elseif beta >= min(Ocline_x,Oaline_x) || beta <= max(Obline_x,Odline_x)
    region=3;
else
    region=2;
end

%% 得到index

left_Ix = max(Ibline_x,Idline_x);%k^{bd}_{in},phi1
right_Ix = min(Ialine_x,Icline_x);%k^{ac}_{in}
right_Ox = min(Oaline_x,Ocline_x);%k^{ac}_{out}
left_Ox = max(Obline_x,Odline_x);%k^{bd}_{out}

if region==1
    
    Center = (left_Ix + right_Ix)/2;
    if Center <= beta && beta <= right_Ix
        index = (right_Ix-beta)/right_Ix;
    else%if Center > beta && beta >= left_Ix
        index = (left_Ix-beta)/left_Ix;
    end
    
else%if region==2
    
    if beta >= right_Ix
        index = (-beta+right_Ix)/(right_Ox-right_Ix);
    else%if beta <= left_Ix
        index = (-beta+left_Ix)/(left_Ox-left_Ix);
    end
     
end
elseif Vx_kmh > 72.5 && Vx_kmh <= 77.5%75
    %% 外边界
for n=1:length(alpharl)
    if abs(alpharl(n))<abs(kekoalphaf)%%鐢ㄤ笉瓒宠浆鍚戞椂鍓嶅悗杞晶鍋忚鐨勫ぇ灏忓叧绯荤瓫閫夊悎閫傜殑
    beta1_right(n)=((sw_angle-kekoalphaf)*lr-lf*alpharl(n))/(lf+lr);
    gamma1_right(n)=((sw_angle-kekoalphaf+alpharl(n))*Vx)/(lf+lr);
    end
end

   beta11_75_right_down=beta1_right(1);
   gamma11_75_right_down=gamma1_right(1);
   beta1n_75_right_up=beta1_right(length(beta1_right));
   gamma1n_75_right_up=gamma1_right(length(gamma1_right));
   
    centerx_75=beta1n_75_right_up-0.0829;
    centery_75=gamma1n_75_right_up-4.3076;
   
    beta1d1_75_left_up=2*centerx_75-beta1_right(1);%鍒╃敤涓偣鍏紡姹傚绉扮偣
    gamma1d1_75_left_up=2*centery_75-gamma1_right(1);%鍒╃敤涓偣鍏紡姹傚绉扮偣
    beta1dn_75_left_down=2*centerx_75-beta1_right(length(beta1_right));%鍒╃敤涓偣鍏紡姹傚绉扮偣
    gamma1dn_75_left_down=2*centery_75-gamma1_right(length(gamma1_right));%鍒╃敤涓偣鍏紡姹傚绉扮偣
    
g1=3.3540+gamma1dn_75_left_down;%璁＄畻ogamma2_down(1)-gamma1dn_75_left_down=锛熶綔涓哄墠闈㈢殑涓�釜鍔犳暟;
b1=0.0571+beta1dn_75_left_down;%obeta2_down(1)-beta1dn_75_left_down=锛�
g2=1.1384+g1;%ogamma2_down(length(ogamma2_down))-ogamma2_down(1)=锛�
b2= 0.0863+b1;%obeta2_down(length(obeta2_down))-obeta2_down(1)=锛�
g3=2*centery_75-g1;%%-g1
b3=2*centerx_75-b1;%%-b1
g4=2*centery_75-g2;%%-g2
b4=2*centerx_75-b2;%%-b2


% x11=gamma1dn_75_left_down:0.000005:g1;
       px111_opposite =       0.01702;
       px112_opposite =       -0.009572;
% x12=g1:0.000005:g2;
       px121_opposite =        -0.173  ;
       px122_opposite =        -0.2843  ;
       px123_opposite =         -0.04049;
       px124_opposite =          0.148;
       px125_opposite =           0.1346 ;
       px126_opposite =       0.03212;
% x13=g2:0.000005:gamma11_75_right_down;
       px131_opposite =    1.049;% (-5.636e+05, -2.701e+05)
       px132_opposite =     -0.1333;% (-6.956e+04, -3.484e+04)
% x21=gamma1d1_75_left_up:0.000005:g4;
       px211_opposite =       1.049 ;
       px212_opposite =         0.1332;
% x22= g4:0.000005:g3;
       px221_opposite =         -0.173   ;% (-6.388e+05, -3.304e+05)
       px222_opposite =          0.2843;% (4.151e+04, 8.218e+04)
       px223_opposite =       -0.04049 ;%  (-561.4, 843.6)
       px224_opposite =        -0.148  ;% (-313, -264.4)
       px225_opposite =          0.1346;%  (18.8, 19.9)
       px226_opposite =        -0.03212;% (-0.3822, -0.3702)
% x23=g3:0.000005:gamma1n_75_right_up;
       px231_opposite =      0.01702;% (-5.636e+05, -2.701e+05)
       px232_opposite =        0.009559;% (-6.956e+04, -3.484e+04)
% x33=gamma11_75_right_down:0.000005:gamma1n_75_right_up;   
       px31_opposite =      -0.0504;%(-21.16, -21.16)
       px32_opposite =       0.3 ;% (2.222, 2.222)
% x44=gamma1dn_75_left_down:0.000005:gamma1d1_75_left_up; 
       px41_opposite =     -0.0504;%(-21.16, -21.16)
       px42_opposite =       -0.3 ;%(-2.222, -2.222)
d3=beta11_75_right_down-px31_opposite*gamma11_75_right_down;
d4=beta1d1_75_left_up-px41_opposite*gamma1d1_75_left_up;
gamma1dn_75_0_opposite= -4.3076;
beta1dn_75_0_opposite=-0.0829;
gamma1d1_75_0_opposite=-0.3942;
beta1d1_75_0_opposite=-0.2801;
       
oobeta1_cal_1 = px111_opposite*(gamma-(gamma1dn_75_left_down(1)-(gamma1dn_75_0_opposite))) + px112_opposite +(beta1dn_75_left_down(1)-(beta1dn_75_0_opposite));
oobeta1_cal = px121_opposite*(gamma-(gamma1dn_75_left_down(1)-(gamma1dn_75_0_opposite))).^5 + px122_opposite*(gamma-(gamma1dn_75_left_down(1)-(gamma1dn_75_0_opposite))).^4 + px123_opposite*(gamma-(gamma1dn_75_left_down(1)-(gamma1dn_75_0_opposite))).^3 + px124_opposite*(gamma-(gamma1dn_75_left_down(1)-(gamma1dn_75_0_opposite))).^2 + px125_opposite*(gamma-(gamma1dn_75_left_down(1)-(gamma1dn_75_0_opposite))) + px126_opposite+(beta1dn_75_left_down(1)-(beta1dn_75_0_opposite));
oobeta1_cal_3 = px131_opposite*(gamma-(gamma1dn_75_left_down(1)-(gamma1dn_75_0_opposite))) + px132_opposite +(beta1dn_75_left_down(1)-(beta1dn_75_0_opposite));
oobeta2_cal_1 = px211_opposite*(gamma-(gamma1d1_75_left_up(1)-(gamma1d1_75_0_opposite))) + px212_opposite +(beta1d1_75_left_up(1)-(beta1d1_75_0_opposite));
oobeta2_cal = px221_opposite*(gamma-(gamma1d1_75_left_up(1)-(gamma1d1_75_0_opposite))).^5 + px222_opposite*(gamma-(gamma1d1_75_left_up(1)-(gamma1d1_75_0_opposite))).^4 + px223_opposite*(gamma-(gamma1d1_75_left_up(1)-(gamma1d1_75_0_opposite))).^3 + px224_opposite*(gamma-(gamma1d1_75_left_up(1)-(gamma1d1_75_0_opposite))).^2 + px225_opposite*(gamma-(gamma1d1_75_left_up(1)-(gamma1d1_75_0_opposite))) + px226_opposite+(beta1d1_75_left_up(1)-(beta1d1_75_0_opposite));
oobeta2_cal_3 = px231_opposite*(gamma-(gamma1d1_75_left_up(1)-(gamma1d1_75_0_opposite))) + px232_opposite +(beta1d1_75_left_up(1)-(beta1d1_75_0_opposite));

Ocline_x = px31_opposite*gamma+d3;
Odline_x = px41_opposite*gamma+d4;

if gamma < g4
    Obline_x = oobeta2_cal_1;
elseif gamma > g3
    Obline_x = oobeta2_cal_3;
else
    Obline_x = oobeta2_cal;
end

if gamma < g1
    Oaline_x = oobeta1_cal_1;
elseif gamma > g2
    Oaline_x = oobeta1_cal_3;
else
    Oaline_x = oobeta1_cal;
end
%% 内边界
gamma1dn_80=gamma1dn_75_left_down+2.8873;
beta1dn_80=beta1dn_75_left_down+0.0450;
gamma11_80=gamma11_75_right_down-0.0594;
beta11_80=beta11_75_right_down-0.1910;
gamma1d1_80=gamma1d1_75_left_up+0.0593;
beta1d1_80=beta1d1_75_left_up+0.1910;
gamma1n_80=gamma1n_75_right_up-2.8874;
beta1n_80=beta1n_75_right_up-0.0450;

px11 =     -0.01488  ;
px12 =      0.08784   ;
px13 =      -0.05734 ;
px21 =       -0.08387 ;
px22 =         0.1758 ;
px23 =       -0.01514  ;
px24 =       -0.1589 ;
px25 =       0.1398;
px26 =     -0.0273 ;
px31 =     0.01488    ;
px32 =      0.08784   ;
px33 =      0.05734 ;
px41 =   -0.08387;
px42 =     -0.1758 ;
px43 =     -0.01514;
px44 =    0.1589  ;
px45 =    0.1398  ;
px46 =   0.0273 ;
px51 =      -0.04725  ;%(-21.16, -21.16)
px52 =     0.105;% (2.222, 2.222)
px61 =      -0.04725  ;%(-21.16, -21.16)
px62 =    -0.105 ;%(-2.222, -2.222)
d5=beta11_80-px51*gamma11_80;
d6=beta1d1_80-px61*gamma1d1_80;

Ibline_x = px21*(gamma-(gamma1d1_80(1)-(-0.3349))).^5 + px22*(gamma-(gamma1d1_80(1)-(-0.3349))).^4 + px23*(gamma-(gamma1d1_80(1)-(-0.3349))).^3 + px24*(gamma-(gamma1d1_80(1)-(-0.3349))).^2 + px25*(gamma-(gamma1d1_80(1)-(-0.3349))) + px26+(beta1d1_80(1)-(-0.0884));
Ialine_x = px41*(gamma-(gamma1dn_80(1)-(-1.4202))).^5 + px42*(gamma-(gamma1dn_80(1)-(-1.4202))).^4 + px43*(gamma-(gamma1dn_80(1)-(-1.4202))).^3 + px44*(gamma-(gamma1dn_80(1)-(-1.4202))).^2 + px45*(gamma-(gamma1dn_80(1)-(-1.4202))) + px46+(beta1dn_80(1)-( -0.0374));
Icline_x = px51*gamma+d5;
Idline_x = px61*gamma+d6;  
%% 判断region
if beta <= min(Icline_x,Ialine_x) && beta >= max(Ibline_x,Idline_x)
    region=1;
elseif beta >= min(Ocline_x,Oaline_x) || beta <= max(Obline_x,Odline_x)
    region=3;
else
    region=2;
end

%% 得到index

left_Ix = max(Ibline_x,Idline_x);%k^{bd}_{in},phi1
right_Ix = min(Ialine_x,Icline_x);%k^{ac}_{in}
right_Ox = min(Oaline_x,Ocline_x);%k^{ac}_{out}
left_Ox = max(Obline_x,Odline_x);%k^{bd}_{out}

if region==1
    
    Center = (left_Ix + right_Ix)/2;
    if Center <= beta && beta <= right_Ix
        index = (right_Ix-beta)/right_Ix;
    else%if Center > beta && beta >= left_Ix
        index = (left_Ix-beta)/left_Ix;
    end
    
else%if region==2
    
    if beta >= right_Ix
        index = (-beta+right_Ix)/(right_Ox-right_Ix);
    else%if beta <= left_Ix
        index = (-beta+left_Ix)/(left_Ox-left_Ix);
    end
     
end
else%if Vx_kmh>77.5 %80
    %% 外边界
for n=1:length(alpharl)
    if abs(alpharl(n))<abs(kekoalphaf)%%鐢ㄤ笉瓒宠浆鍚戞椂鍓嶅悗杞晶鍋忚鐨勫ぇ灏忓叧绯荤瓫閫夊悎閫傜殑
    beta1_right(n)=((sw_angle-kekoalphaf)*lr-lf*alpharl(n))/(lf+lr);
    gamma1_right(n)=((sw_angle-kekoalphaf+alpharl(n))*Vx)/(lf+lr);
    end
end

   beta11_80_right_down=beta1_right(1);
   gamma11_80_right_down=gamma1_right(1);
   beta1n_80_right_up=beta1_right(length(beta1_right));
   gamma1n_80_right_up=gamma1_right(length(gamma1_right));
   
    centerx_80=beta1n_80_right_up-0.0829;
    centery_80=gamma1n_80_right_up-4.5948;
   
    beta1d1_80_left_up=2*centerx_80-beta1_right(1);%鍒╃敤涓偣鍏紡姹傚绉扮偣
    gamma1d1_80_left_up=2*centery_80-gamma1_right(1);%鍒╃敤涓偣鍏紡姹傚绉扮偣
    beta1dn_80_left_down=2*centerx_80-beta1_right(length(beta1_right));%鍒╃敤涓偣鍏紡姹傚绉扮偣
    gamma1dn_80_left_down=2*centery_80-gamma1_right(length(gamma1_right));%鍒╃敤涓偣鍏紡姹傚绉扮偣
    
g1=3.5776+gamma1dn_80_left_down;%璁＄畻ogamma2_down(1)-gamma1dn_80_left_down=锛熶綔涓哄墠闈㈢殑涓�釜鍔犳暟;
b1=0.0571+beta1dn_80_left_down;%obeta2_down(1)-beta1dn_80_left_down=锛�
g2= 1.2143+g1;%ogamma2_down(length(ogamma2_down))-ogamma2_down(1)=锛�
b2= 0.0863+b1;%obeta2_down(length(obeta2_down))-obeta2_down(1)=锛�
g3=2*centery_80-g1;%%-g1
b3=2*centerx_80-b1;%%-b1
g4=2*centery_80-g2;%%-g2
b4=2*centerx_80-b2;%%-b2


% x11=gamma1dn_80_left_down:0.000005:g1;
       px111_opposite =       0.01596;
       px112_opposite =       -0.009571;
% x12=g1:0.000005:g2;
       px121_opposite =        -0.2259  ;
       px122_opposite =        -0.41  ;
       px123_opposite =          -0.1224  ;
       px124_opposite =         0.1398;
       px125_opposite =           0.1343  ;
       px126_opposite =         0.03137;
% x13=g2:0.000005:gamma11_80_right_down;
       px131_opposite =    0.9829;% (-5.636e+05, -2.701e+05)
       px132_opposite =     -0.1333;% (-6.956e+04, -3.484e+04)
% x21=gamma1d1_80_left_up:0.000005:g4;
       px211_opposite =        0.9829;
       px212_opposite =         0.1332;
% x22= g4:0.000005:g3;
       px221_opposite =         -0.2259  ;% (-6.388e+05, -3.304e+05)
       px222_opposite =           0.41;% (4.151e+04, 8.218e+04)
       px223_opposite =      -0.1224 ;%  (-561.4, 843.6)
       px224_opposite =       -0.1398 ;% (-313, -264.4)
       px225_opposite =          0.1343 ;%  (18.8, 19.9)
       px226_opposite =          -0.03137;% (-0.3822, -0.3702)
% x23=g3:0.000005:gamma1n_80_right_up;
       px231_opposite =        0.01596;% (-5.636e+05, -2.701e+05)
       px232_opposite =       0.009559;% (-6.956e+04, -3.484e+04)
% x33=gamma11_80_right_down:0.000005:gamma1n_80_right_up;   
       px31_opposite =       -0.04725;%(-21.16, -21.16)
       px32_opposite =       0.3 ;% (2.222, 2.222)
% x44=gamma1dn_80_left_down:0.000005:gamma1d1_80_left_up; 
       px41_opposite =     -0.04725;%(-21.16, -21.16)
       px42_opposite =       -0.3 ;%(-2.222, -2.222)
d3=beta11_80_right_down-px31_opposite*gamma11_80_right_down;
d4=beta1d1_80_left_up-px41_opposite*gamma1d1_80_left_up;
gamma1dn_80_0_opposite= -4.5948;
beta1dn_80_0_opposite=-0.0829;
gamma1d1_80_0_opposite=-0.4205;
beta1d1_80_0_opposite=-0.2801;
       
oobeta1_cal_1 = px111_opposite*(gamma-(gamma1dn_80_left_down(1)-(gamma1dn_80_0_opposite))) + px112_opposite +(beta1dn_80_left_down(1)-(beta1dn_80_0_opposite));
oobeta1_cal = px121_opposite*(gamma-(gamma1dn_80_left_down(1)-(gamma1dn_80_0_opposite))).^5 + px122_opposite*(gamma-(gamma1dn_80_left_down(1)-(gamma1dn_80_0_opposite))).^4 + px123_opposite*(gamma-(gamma1dn_80_left_down(1)-(gamma1dn_80_0_opposite))).^3 + px124_opposite*(gamma-(gamma1dn_80_left_down(1)-(gamma1dn_80_0_opposite))).^2 + px125_opposite*(gamma-(gamma1dn_80_left_down(1)-(gamma1dn_80_0_opposite))) + px126_opposite+(beta1dn_80_left_down(1)-(beta1dn_80_0_opposite));
oobeta1_cal_3 = px131_opposite*(gamma-(gamma1dn_80_left_down(1)-(gamma1dn_80_0_opposite))) + px132_opposite +(beta1dn_80_left_down(1)-(beta1dn_80_0_opposite));
oobeta2_cal_1 = px211_opposite*(gamma-(gamma1d1_80_left_up(1)-(gamma1d1_80_0_opposite))) + px212_opposite +(beta1d1_80_left_up(1)-(beta1d1_80_0_opposite));
oobeta2_cal = px221_opposite*(gamma-(gamma1d1_80_left_up(1)-(gamma1d1_80_0_opposite))).^5 + px222_opposite*(gamma-(gamma1d1_80_left_up(1)-(gamma1d1_80_0_opposite))).^4 + px223_opposite*(gamma-(gamma1d1_80_left_up(1)-(gamma1d1_80_0_opposite))).^3 + px224_opposite*(gamma-(gamma1d1_80_left_up(1)-(gamma1d1_80_0_opposite))).^2 + px225_opposite*(gamma-(gamma1d1_80_left_up(1)-(gamma1d1_80_0_opposite))) + px226_opposite+(beta1d1_80_left_up(1)-(beta1d1_80_0_opposite));
oobeta2_cal_3 = px231_opposite*(gamma-(gamma1d1_80_left_up(1)-(gamma1d1_80_0_opposite))) + px232_opposite +(beta1d1_80_left_up(1)-(beta1d1_80_0_opposite));

Ocline_x = px31_opposite*gamma+d3;
Odline_x = px41_opposite*gamma+d4;

if gamma < g4
    Obline_x = oobeta2_cal_1;
elseif gamma > g3
    Obline_x = oobeta2_cal_3;
else
    Obline_x = oobeta2_cal;
end

if gamma < g1
    Oaline_x = oobeta1_cal_1;
elseif gamma > g2
    Oaline_x = oobeta1_cal_3;
else
    Oaline_x = oobeta1_cal;
end
%% 内边界
gamma1dn_80=gamma1dn_80_left_down+3.1746;
beta1dn_80=beta1dn_80_left_down+0.0450;
gamma11_80=gamma11_80_right_down-0.0857;
beta11_80=beta11_80_right_down-0.1910;
gamma1d1_80=gamma1d1_80_left_up+0.0856;
beta1d1_80=beta1d1_80_left_up+0.1910;
gamma1n_80=gamma1n_80_right_up -3.1746;
beta1n_80=beta1n_80_right_up-0.0450;

px21 =       -0.06186;
px22 =        0.1208 ;
px23 =         0.025  ;
px24 =        -0.1639 ;
px25 =      0.1329;
px26 =       -0.02599;
px41 =    -0.06186 ;
px42 =    -0.1208 ;
px43 =      0.025;
px44 =     0.1639  ;
px45 =    0.1329  ;
px46 =     0.02599 ;
px51 =    -0.04725 ;%(-21.16, -21.16)
px52 =          0.105 ;% (2.222, 2.222)
px61 =    -0.04725  ;%(-21.16, -21.16)
px62 =    -0.105 ;%(-2.222, -2.222)
d5=beta11_80-px51*gamma11_80;
d6=beta1d1_80-px61*gamma1d1_80;

Ibline_x = px21*(gamma-(gamma1d1_80(1)-(-0.3349))).^5 + px22*(gamma-(gamma1d1_80(1)-(-0.3349))).^4 + px23*(gamma-(gamma1d1_80(1)-(-0.3349))).^3 + px24*(gamma-(gamma1d1_80(1)-(-0.3349))).^2 + px25*(gamma-(gamma1d1_80(1)-(-0.3349))) + px26+(beta1d1_80(1)-(-0.0882));
Ialine_x = px41*(gamma-(gamma1dn_80(1)-(-1.4202))).^5 + px42*(gamma-(gamma1dn_80(1)-(-1.4202))).^4 + px43*(gamma-(gamma1dn_80(1)-(-1.4202))).^3 + px44*(gamma-(gamma1dn_80(1)-(-1.4202))).^2 + px45*(gamma-(gamma1dn_80(1)-(-1.4202))) + px46+(beta1dn_80(1)-( -0.0373));
Icline_x = px51*gamma+d5;
Idline_x = px61*gamma+d6;


%% 判断region
if beta <= min(Icline_x,Ialine_x) && beta >= max(Ibline_x,Idline_x)
    region=1;
elseif beta >= min(Ocline_x,Oaline_x) || beta <= max(Obline_x,Odline_x)
    region=3;
else
    region=2;
end

%% 得到index

left_Ix = max(Ibline_x,Idline_x);%k^{bd}_{in},phi1
right_Ix = min(Ialine_x,Icline_x);%k^{ac}_{in}
right_Ox = min(Oaline_x,Ocline_x);%k^{ac}_{out}
left_Ox = max(Obline_x,Odline_x);%k^{bd}_{out}

if region==1
    
    Center = (left_Ix + right_Ix)/2;
    if Center <= beta && beta <= right_Ix
        index = (right_Ix-beta)/right_Ix;
    else%if Center > beta && beta >= left_Ix
        index = (left_Ix-beta)/left_Ix;
    end
    
else%if region==2
    
    if beta >= right_Ix
        index = (-beta+right_Ix)/(right_Ox-right_Ix);
    else%if beta <= left_Ix
        index = (-beta+left_Ix)/(left_Ox-left_Ix);
    end
     
end
end

if region==1
 index
    
else%if region==2
    
    if beta >= right_Ix
        index = (-beta+right_Ix)/(right_Ox-right_Ix);
    else%if beta <= left_Ix
        index = (-beta+left_Ix)/(left_Ox-left_Ix);
    end
     
end
end
